simulink model "RadSimulink"  (R2020a)
settings: Solver=VariableStepAuto  StartTime=0.0  StopTime=10.0  RelTol=1e-3
values from neighbouring files (symbols this model uses):
  cz = str2num(get(handles.edit2,'string'))    [GUI.m]
  pz = str2num(get(handles.edit1,'string'))    [GUI.m]
  ti = str2num(get(handles.edit5,'string'))    [GUI.m]
  tp = str2num(get(handles.edit4,'string'))    [GUI.m]
  zl = str2num(get(handles.edit3,'string'))    [GUI.m]
libraries: neural x206, fuzblock x2
(part 2 of 3)

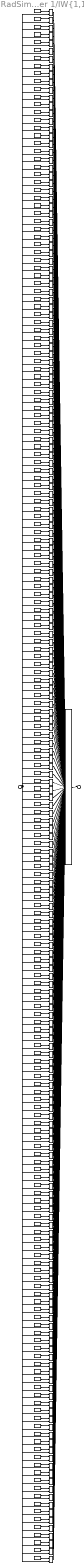
== system RadSimulink/Function Fitting Neural Network/Layer 1/IW{1,1} ==
  "pd{1,1}" : Inport  PortDimensions=5
      mask Display: e = 0.06;c1 = [120 230 180]/255;c2 = ([120 230 180]+0)/(256+128);c3 = ([120 230 180]+128)/(256+128);patch([0 1 1 0],[0 0 1 1],c1);patch([0 1 1 1-e 1-e 0+e],[0 0 1 1-e 0+e 0+e],c2);patch([0 0 1 1-e 0+e 0+e],[0 1 1 1-e 1-e 0+e],c3);plot([0 1 1 0 0],[0 0 1 1 0]);
  "IW{1,1}(1,:)'" : Constant  Value=[-1.1024971237361669285093057624180801212787628173828125;-2.42025893729763996731207953416742384433746337890625;-0.1951758632417351646548553389948210678994655609130859375;-1.7662876637968849546922456283937208354473114013671875;-2.01734664909667760213096698862500488758087158203125]
      mask Display: e = 0.06;c1 = [120 150 230]/255;c2 = ([120 150 230]+0)/383;c3 = ([120 150 230]+128)/383;patch([0 1 1 0],[0 0 1 1],c1);patch([0 1 1 1-e 1-e 0+e],[0 0 1 1-e 0+e 0+e],c2);patch([0 0 1 1-e 0+e 0+e],[0 1 1 1-e 1-e 0+e],c3);plot([0 1 1 0 0],[0 0 1 1 0]);disp('Weights');
  "IW{1,1}(10,:)'" : Constant  Value=[2.101523545932024727989073653589002788066864013671875;-1.7279665023119312738941744100884534418582916259765625;1.1178691452224647218116615476901642978191375732421875;-0.27934657220397907106956836287281475961208343505859375;2.880254256165533544020718181855045258998870849609375]
      mask Display: e = 0.06;c1 = [120 150 230]/255;c2 = ([120 150 230]+0)/383;c3 = ([120 150 230]+128)/383;patch([0 1 1 0],[0 0 1 1],c1);patch([0 1 1 1-e 1-e 0+e],[0 0 1 1-e 0+e 0+e],c2);patch([0 0 1 1-e 0+e 0+e],[0 1 1 1-e 1-e 0+e],c3);plot([0 1 1 0 0],[0 0 1 1 0]);disp('Weights');
  "IW{1,1}(100,:)'" : Constant  Value=[-1.0080768381000433375760394483222626149654388427734375;0.06504466674938051695686880293578724376857280731201171875;-2.437083695314801179421237975475378334522247314453125;-0.60085262232023317618967439557309262454509735107421875;2.912213889031785907235416743787936866283416748046875]
      mask Display: e = 0.06;c1 = [120 150 230]/255;c2 = ([120 150 230]+0)/383;c3 = ([120 150 230]+128)/383;patch([0 1 1 0],[0 0 1 1],c1);patch([0 1 1 1-e 1-e 0+e],[0 0 1 1-e 0+e 0+e],c2);patch([0 0 1 1-e 0+e 0+e],[0 1 1 1-e 1-e 0+e],c3);plot([0 1 1 0 0],[0 0 1 1 0]);disp('Weights');
  "IW{1,1}(101,:)'" : Constant  Value=[1.90336093057931687866357606253586709499359130859375;-1.126709319667938746789559445460326969623565673828125;-2.31817597529505636799740386777557432651519775390625;1.6272516351571402193343374165124259889125823974609375;-1.368723252103397403089957151678390800952911376953125]
      mask Display: e = 0.06;c1 = [120 150 230]/255;c2 = ([120 150 230]+0)/383;c3 = ([120 150 230]+128)/383;patch([0 1 1 0],[0 0 1 1],c1);patch([0 1 1 1-e 1-e 0+e],[0 0 1 1-e 0+e 0+e],c2);patch([0 0 1 1-e 0+e 0+e],[0 1 1 1-e 1-e 0+e],c3);plot([0 1 1 0 0],[0 0 1 1 0]);disp('Weights');
  "IW{1,1}(102,:)'" : Constant  Value=[-3.420026756921864308225167405907995998859405517578125;-2.3719950536146399144854512996971607208251953125;1.1313743416636159455634924597688950598239898681640625;-0.8552105117849888582526318714371882379055023193359375;0.233304600818531604478067720265244133770465850830078125]
      mask Display: e = 0.06;c1 = [120 150 230]/255;c2 = ([120 150 230]+0)/383;c3 = ([120 150 230]+128)/383;patch([0 1 1 0],[0 0 1 1],c1);patch([0 1 1 1-e 1-e 0+e],[0 0 1 1-e 0+e 0+e],c2);patch([0 0 1 1-e 0+e 0+e],[0 1 1 1-e 1-e 0+e],c3);plot([0 1 1 0 0],[0 0 1 1 0]);disp('Weights');
  "IW{1,1}(103,:)'" : Constant  Value=[-0.7245749152369149737040743275429122149944305419921875;2.719538996825153542857833599555306136608123779296875;-0.34034567501443147019557500243536196649074554443359375;-2.62175331828034519077164077316410839557647705078125;-1.79375045778324260226099795545451343059539794921875]
      mask Display: e = 0.06;c1 = [120 150 230]/255;c2 = ([120 150 230]+0)/383;c3 = ([120 150 230]+128)/383;patch([0 1 1 0],[0 0 1 1],c1);patch([0 1 1 1-e 1-e 0+e],[0 0 1 1-e 0+e 0+e],c2);patch([0 0 1 1-e 0+e 0+e],[0 1 1 1-e 1-e 0+e],c3);plot([0 1 1 0 0],[0 0 1 1 0]);disp('Weights');
  "IW{1,1}(104,:)'" : Constant  Value=[-1.8276546952938861334558851012843661010265350341796875;3.1424452420276391961806439212523400783538818359375;2.819758895819064914434193269698880612850189208984375;-0.10000487520686705822381412644972442649304866790771484375;0.88030108858768307822373344606603495776653289794921875]
      mask Display: e = 0.06;c1 = [120 150 230]/255;c2 = ([120 150 230]+0)/383;c3 = ([120 150 230]+128)/383;patch([0 1 1 0],[0 0 1 1],c1);patch([0 1 1 1-e 1-e 0+e],[0 0 1 1-e 0+e 0+e],c2);patch([0 0 1 1-e 0+e 0+e],[0 1 1 1-e 1-e 0+e],c3);plot([0 1 1 0 0],[0 0 1 1 0]);disp('Weights');
  "IW{1,1}(105,:)'" : Constant  Value=[-1.955119046550140016194063719012774527072906494140625;2.26029192919587718080265403841622173786163330078125;-0.84774494451610082901282794409780763089656829833984375;-0.38953484467059806828359569408348761498928070068359375;2.197168941225040583731242804788053035736083984375]
      mask Display: e = 0.06;c1 = [120 150 230]/255;c2 = ([120 150 230]+0)/383;c3 = ([120 150 230]+128)/383;patch([0 1 1 0],[0 0 1 1],c1);patch([0 1 1 1-e 1-e 0+e],[0 0 1 1-e 0+e 0+e],c2);patch([0 0 1 1-e 0+e 0+e],[0 1 1 1-e 1-e 0+e],c3);plot([0 1 1 0 0],[0 0 1 1 0]);disp('Weights');
  "IW{1,1}(106,:)'" : Constant  Value=[-2.32279050408599641031059945817105472087860107421875;0.94744858728796532698623877877253107726573944091796875;-1.5499805306115224112772921216674149036407470703125;2.097487556649907158856649402878247201442718505859375;-1.791807377519587074488072175881825387477874755859375]
      mask Display: e = 0.06;c1 = [120 150 230]/255;c2 = ([120 150 230]+0)/383;c3 = ([120 150 230]+128)/383;patch([0 1 1 0],[0 0 1 1],c1);patch([0 1 1 1-e 1-e 0+e],[0 0 1 1-e 0+e 0+e],c2);patch([0 0 1 1-e 0+e 0+e],[0 1 1 1-e 1-e 0+e],c3);plot([0 1 1 0 0],[0 0 1 1 0]);disp('Weights');
  "IW{1,1}(107,:)'" : Constant  Value=[1.1809257823517860241935295562143437564373016357421875;-2.377719411022709561365218178252689540386199951171875;0.2141296858350458520714454380140523426234722137451171875;-1.1815675916247567744932212008279748260974884033203125;2.70168779430114813777663584914989769458770751953125]
      mask Display: e = 0.06;c1 = [120 150 230]/255;c2 = ([120 150 230]+0)/383;c3 = ([120 150 230]+128)/383;patch([0 1 1 0],[0 0 1 1],c1);patch([0 1 1 1-e 1-e 0+e],[0 0 1 1-e 0+e 0+e],c2);patch([0 0 1 1-e 0+e 0+e],[0 1 1 1-e 1-e 0+e],c3);plot([0 1 1 0 0],[0 0 1 1 0]);disp('Weights');
  "IW{1,1}(108,:)'" : Constant  Value=[-1.754914904257402152865097377798520028591156005859375;-2.0911361399005361505487599060870707035064697265625;2.542284700714983358693643822334706783294677734375;1.9958867986801454019740731382626108825206756591796875;-1.67034476062302683629923194530420005321502685546875]
      mask Display: e = 0.06;c1 = [120 150 230]/255;c2 = ([120 150 230]+0)/383;c3 = ([120 150 230]+128)/383;patch([0 1 1 0],[0 0 1 1],c1);patch([0 1 1 1-e 1-e 0+e],[0 0 1 1-e 0+e 0+e],c2);patch([0 0 1 1-e 0+e 0+e],[0 1 1 1-e 1-e 0+e],c3);plot([0 1 1 0 0],[0 0 1 1 0]);disp('Weights');
  "IW{1,1}(109,:)'" : Constant  Value=[0.956521745717475280201824716641567647457122802734375;-2.50335089270634636449130994151346385478973388671875;1.2037065443916625806508591267629526555538177490234375;0.60555610759611766535925880816648714244365692138671875;-2.731580459628556667439625016413629055023193359375]
      mask Display: e = 0.06;c1 = [120 150 230]/255;c2 = ([120 150 230]+0)/383;c3 = ([120 150 230]+128)/383;patch([0 1 1 0],[0 0 1 1],c1);patch([0 1 1 1-e 1-e 0+e],[0 0 1 1-e 0+e 0+e],c2);patch([0 0 1 1-e 0+e 0+e],[0 1 1 1-e 1-e 0+e],c3);plot([0 1 1 0 0],[0 0 1 1 0]);disp('Weights');
  "IW{1,1}(11,:)'" : Constant  Value=[-2.907949635275226540898074745200574398040771484375;1.1530656903068148277924365174840204417705535888671875;-0.443569230139339631957540177609189413487911224365234375;1.4059497597816703606810051496722735464572906494140625;2.099149397548405460156573099084198474884033203125]
      mask Display: e = 0.06;c1 = [120 150 230]/255;c2 = ([120 150 230]+0)/383;c3 = ([120 150 230]+128)/383;patch([0 1 1 0],[0 0 1 1],c1);patch([0 1 1 1-e 1-e 0+e],[0 0 1 1-e 0+e 0+e],c2);patch([0 0 1 1-e 0+e 0+e],[0 1 1 1-e 1-e 0+e],c3);plot([0 1 1 0 0],[0 0 1 1 0]);disp('Weights');
  "IW{1,1}(110,:)'" : Constant  Value=[-1.6020415711927344926124305857229046523571014404296875;-3.0917400563691845860603280016221106052398681640625;-0.9714288758683198299337391290464438498020172119140625;-2.2679764643333104601197192096151411533355712890625;0.669326600522941905779816806898452341556549072265625]
      mask Display: e = 0.06;c1 = [120 150 230]/255;c2 = ([120 150 230]+0)/383;c3 = ([120 150 230]+128)/383;patch([0 1 1 0],[0 0 1 1],c1);patch([0 1 1 1-e 1-e 0+e],[0 0 1 1-e 0+e 0+e],c2);patch([0 0 1 1-e 0+e 0+e],[0 1 1 1-e 1-e 0+e],c3);plot([0 1 1 0 0],[0 0 1 1 0]);disp('Weights');
  "IW{1,1}(111,:)'" : Constant  Value=[1.162354455160433897020766380592249333858489990234375;1.5263583187996536683073145468370057642459869384765625;-1.9318884103074271951783202894148416817188262939453125;-1.7446165484139708468092067050747573375701904296875;-2.8400204539045343921088715433143079280853271484375]
      mask Display: e = 0.06;c1 = [120 150 230]/255;c2 = ([120 150 230]+0)/383;c3 = ([120 150 230]+128)/383;patch([0 1 1 0],[0 0 1 1],c1);patch([0 1 1 1-e 1-e 0+e],[0 0 1 1-e 0+e 0+e],c2);patch([0 0 1 1-e 0+e 0+e],[0 1 1 1-e 1-e 0+e],c3);plot([0 1 1 0 0],[0 0 1 1 0]);disp('Weights');
  "IW{1,1}(112,:)'" : Constant  Value=[0.66765089953219725060762357315979897975921630859375;-1.9914835830233432734104326300439424812793731689453125;1.8164696639128068422763817579834721982479095458984375;0.2068577426128505869495910474142874591052532196044921875;-3.01193773462074698699098007637076079845428466796875]
      mask Display: e = 0.06;c1 = [120 150 230]/255;c2 = ([120 150 230]+0)/383;c3 = ([120 150 230]+128)/383;patch([0 1 1 0],[0 0 1 1],c1);patch([0 1 1 1-e 1-e 0+e],[0 0 1 1-e 0+e 0+e],c2);patch([0 0 1 1-e 0+e 0+e],[0 1 1 1-e 1-e 0+e],c3);plot([0 1 1 0 0],[0 0 1 1 0]);disp('Weights');
  "IW{1,1}(113,:)'" : Constant  Value=[-1.3410265394460332277759562202845700085163116455078125;1.4528723409373867081484377195010893046855926513671875;4.09747304901806597143831822904758155345916748046875;0.5194580229380536540162438541301526129245758056640625;1.6134633116029968302740371655090712010860443115234375]
      mask Display: e = 0.06;c1 = [120 150 230]/255;c2 = ([120 150 230]+0)/383;c3 = ([120 150 230]+128)/383;patch([0 1 1 0],[0 0 1 1],c1);patch([0 1 1 1-e 1-e 0+e],[0 0 1 1-e 0+e 0+e],c2);patch([0 0 1 1-e 0+e 0+e],[0 1 1 1-e 1-e 0+e],c3);plot([0 1 1 0 0],[0 0 1 1 0]);disp('Weights');
  "IW{1,1}(114,:)'" : Constant  Value=[2.19775277811335367772471727221272885799407958984375;1.530445614021247013880611120839603245258331298828125;-0.51276813648967511927168061447446234524250030517578125;-1.439648029384903882288426757440902292728424072265625;-3.040338611642841026849737318116240203380584716796875]
      mask Display: e = 0.06;c1 = [120 150 230]/255;c2 = ([120 150 230]+0)/383;c3 = ([120 150 230]+128)/383;patch([0 1 1 0],[0 0 1 1],c1);patch([0 1 1 1-e 1-e 0+e],[0 0 1 1-e 0+e 0+e],c2);patch([0 0 1 1-e 0+e 0+e],[0 1 1 1-e 1-e 0+e],c3);plot([0 1 1 0 0],[0 0 1 1 0]);disp('Weights');
  "IW{1,1}(115,:)'" : Constant  Value=[1.8961919249288563538158314258907921612262725830078125;0.41129351010530157406464013547520153224468231201171875;-2.248095539210364979254563877475447952747344970703125;-1.3547463652555962188017701919307000935077667236328125;2.75720385899369802018554764799773693084716796875]
      mask Display: e = 0.06;c1 = [120 150 230]/255;c2 = ([120 150 230]+0)/383;c3 = ([120 150 230]+128)/383;patch([0 1 1 0],[0 0 1 1],c1);patch([0 1 1 1-e 1-e 0+e],[0 0 1 1-e 0+e 0+e],c2);patch([0 0 1 1-e 0+e 0+e],[0 1 1 1-e 1-e 0+e],c3);plot([0 1 1 0 0],[0 0 1 1 0]);disp('Weights');
  "IW{1,1}(116,:)'" : Constant  Value=[2.954413030926638317197330252383835613727569580078125;-0.88633584372641716075946760611259378492832183837890625;-2.12033955906994986406743919360451400279998779296875;1.76130835936309804168331538676284253597259521484375;-0.1357983118735323901926648204607772640883922576904296875]
      mask Display: e = 0.06;c1 = [120 150 230]/255;c2 = ([120 150 230]+0)/383;c3 = ([120 150 230]+128)/383;patch([0 1 1 0],[0 0 1 1],c1);patch([0 1 1 1-e 1-e 0+e],[0 0 1 1-e 0+e 0+e],c2);patch([0 0 1 1-e 0+e 0+e],[0 1 1 1-e 1-e 0+e],c3);plot([0 1 1 0 0],[0 0 1 1 0]);disp('Weights');
  "IW{1,1}(117,:)'" : Constant  Value=[-4.02991069960216474754588489304296672344207763671875;1.9833370043181337560866950298077426850795745849609375;0.046775997960406622000473220168714760802686214447021484375;0.734776445964431701440844335593283176422119140625;-0.89640460868724025633724750150577165186405181884765625]
      mask Display: e = 0.06;c1 = [120 150 230]/255;c2 = ([120 150 230]+0)/383;c3 = ([120 150 230]+128)/383;patch([0 1 1 0],[0 0 1 1],c1);patch([0 1 1 1-e 1-e 0+e],[0 0 1 1-e 0+e 0+e],c2);patch([0 0 1 1-e 0+e 0+e],[0 1 1 1-e 1-e 0+e],c3);plot([0 1 1 0 0],[0 0 1 1 0]);disp('Weights');
  "IW{1,1}(118,:)'" : Constant  Value=[0.69244616119575308488265363848768174648284912109375;-1.6956716845926533832056293249479494988918304443359375;-2.57710351212775901075247020344249904155731201171875;-2.702734985715044668808104688650928437709808349609375;1.1181759860109174997688796793227083981037139892578125]
      mask Display: e = 0.06;c1 = [120 150 230]/255;c2 = ([120 150 230]+0)/383;c3 = ([120 150 230]+128)/383;patch([0 1 1 0],[0 0 1 1],c1);patch([0 1 1 1-e 1-e 0+e],[0 0 1 1-e 0+e 0+e],c2);patch([0 0 1 1-e 0+e 0+e],[0 1 1 1-e 1-e 0+e],c3);plot([0 1 1 0 0],[0 0 1 1 0]);disp('Weights');
  "IW{1,1}(119,:)'" : Constant  Value=[-2.737537295445146678929404515656642615795135498046875;-0.81241155860551350631482137032435275614261627197265625;-1.0933153794961827376397422995069064199924468994140625;1.143052193414451966901879131910391151905059814453125;2.879019332145628329300279801827855408191680908203125]
      mask Display: e = 0.06;c1 = [120 150 230]/255;c2 = ([120 150 230]+0)/383;c3 = ([120 150 230]+128)/383;patch([0 1 1 0],[0 0 1 1],c1);patch([0 1 1 1-e 1-e 0+e],[0 0 1 1-e 0+e 0+e],c2);patch([0 0 1 1-e 0+e 0+e],[0 1 1 1-e 1-e 0+e],c3);plot([0 1 1 0 0],[0 0 1 1 0]);disp('Weights');
  "IW{1,1}(12,:)'" : Constant  Value=[-1.8135943539993935047505146940238773822784423828125;-3.103634828364266073918997790315188467502593994140625;-0.301922130932056387297990340812248177826404571533203125;-0.1237979411920113459455450310997548513114452362060546875;-1.41910702071063798967998081934638321399688720703125]
      mask Display: e = 0.06;c1 = [120 150 230]/255;c2 = ([120 150 230]+0)/383;c3 = ([120 150 230]+128)/383;patch([0 1 1 0],[0 0 1 1],c1);patch([0 1 1 1-e 1-e 0+e],[0 0 1 1-e 0+e 0+e],c2);patch([0 0 1 1-e 0+e 0+e],[0 1 1 1-e 1-e 0+e],c3);plot([0 1 1 0 0],[0 0 1 1 0]);disp('Weights');
  "IW{1,1}(120,:)'" : Constant  Value=[-3.34213975887307146450666550663299858570098876953125;2.790486751775154150578828193829394876956939697265625;-0.302405210762672016500118843396194279193878173828125;-0.257404953550620929636494338410557247698307037353515625;-0.2017369321757929989669122505802079103887081146240234375]
      mask Display: e = 0.06;c1 = [120 150 230]/255;c2 = ([120 150 230]+0)/383;c3 = ([120 150 230]+128)/383;patch([0 1 1 0],[0 0 1 1],c1);patch([0 1 1 1-e 1-e 0+e],[0 0 1 1-e 0+e 0+e],c2);patch([0 0 1 1-e 0+e 0+e],[0 1 1 1-e 1-e 0+e],c3);plot([0 1 1 0 0],[0 0 1 1 0]);disp('Weights');
  "IW{1,1}(121,:)'" : Constant  Value=[-3.392294521732422740711854203254915773868560791015625;0.20942239687643027234997816776740364730358123779296875;-1.3125370002407936720345560388523153960704803466796875;-0.14378919640720833061919847750687040388584136962890625;2.228432434247277882377602509222924709320068359375]
      mask Display: e = 0.06;c1 = [120 150 230]/255;c2 = ([120 150 230]+0)/383;c3 = ([120 150 230]+128)/383;patch([0 1 1 0],[0 0 1 1],c1);patch([0 1 1 1-e 1-e 0+e],[0 0 1 1-e 0+e 0+e],c2);patch([0 0 1 1-e 0+e 0+e],[0 1 1 1-e 1-e 0+e],c3);plot([0 1 1 0 0],[0 0 1 1 0]);disp('Weights');
  "IW{1,1}(122,:)'" : Constant  Value=[-1.75905539540671629339385617640800774097442626953125;-3.187451027508598766502245780429802834987640380859375;-1.645529519450947386616235235123895108699798583984375;2.67049482505225466155707181314937770366668701171875;0.7503515450185374024982820628792978823184967041015625]
      mask Display: e = 0.06;c1 = [120 150 230]/255;c2 = ([120 150 230]+0)/383;c3 = ([120 150 230]+128)/383;patch([0 1 1 0],[0 0 1 1],c1);patch([0 1 1 1-e 1-e 0+e],[0 0 1 1-e 0+e 0+e],c2);patch([0 0 1 1-e 0+e 0+e],[0 1 1 1-e 1-e 0+e],c3);plot([0 1 1 0 0],[0 0 1 1 0]);disp('Weights');
  "IW{1,1}(123,:)'" : Constant  Value=[-2.788792847496659899064752607955597341060638427734375;1.6776656245569110392779066387447528541088104248046875;-0.304824112680752212778401144532836042344570159912109375;-1.2160626373394511912096049854881130158901214599609375;2.776459447970099692071244135149754583835601806640625]
      mask Display: e = 0.06;c1 = [120 150 230]/255;c2 = ([120 150 230]+0)/383;c3 = ([120 150 230]+128)/383;patch([0 1 1 0],[0 0 1 1],c1);patch([0 1 1 1-e 1-e 0+e],[0 0 1 1-e 0+e 0+e],c2);patch([0 0 1 1-e 0+e 0+e],[0 1 1 1-e 1-e 0+e],c3);plot([0 1 1 0 0],[0 0 1 1 0]);disp('Weights');
  "IW{1,1}(124,:)'" : Constant  Value=[-0.80664229937318487895225871397997252643108367919921875;-2.19903462899787793816130943014286458492279052734375;-1.4063350337747901885876444794121198356151580810546875;-2.9997677450250908037787667126394808292388916015625;0.331515823929653230539571495683048851788043975830078125]
      mask Display: e = 0.06;c1 = [120 150 230]/255;c2 = ([120 150 230]+0)/383;c3 = ([120 150 230]+128)/383;patch([0 1 1 0],[0 0 1 1],c1);patch([0 1 1 1-e 1-e 0+e],[0 0 1 1-e 0+e 0+e],c2);patch([0 0 1 1-e 0+e 0+e],[0 1 1 1-e 1-e 0+e],c3);plot([0 1 1 0 0],[0 0 1 1 0]);disp('Weights');
  "IW{1,1}(125,:)'" : Constant  Value=[-1.2121170429702983195596743826172314584255218505859375;2.16495630448694864611525190412066876888275146484375;-2.124413283432712962195410000276751816272735595703125;-2.12457525827358661985044818720780313014984130859375;-0.67667681596699591484167513044667430222034454345703125]
      mask Display: e = 0.06;c1 = [120 150 230]/255;c2 = ([120 150 230]+0)/383;c3 = ([120 150 230]+128)/383;patch([0 1 1 0],[0 0 1 1],c1);patch([0 1 1 1-e 1-e 0+e],[0 0 1 1-e 0+e 0+e],c2);patch([0 0 1 1-e 0+e 0+e],[0 1 1 1-e 1-e 0+e],c3);plot([0 1 1 0 0],[0 0 1 1 0]);disp('Weights');
  "IW{1,1}(126,:)'" : Constant  Value=[-0.7999665946026801588430998890544287860393524169921875;-2.048714130895408658261658274568617343902587890625;1.4521789817209083128801694329013116657733917236328125;0.9816305616312812620805061669670976698398590087890625;3.159907850832450293410147423855960369110107421875]
      mask Display: e = 0.06;c1 = [120 150 230]/255;c2 = ([120 150 230]+0)/383;c3 = ([120 150 230]+128)/383;patch([0 1 1 0],[0 0 1 1],c1);patch([0 1 1 1-e 1-e 0+e],[0 0 1 1-e 0+e 0+e],c2);patch([0 0 1 1-e 0+e 0+e],[0 1 1 1-e 1-e 0+e],c3);plot([0 1 1 0 0],[0 0 1 1 0]);disp('Weights');
  "IW{1,1}(127,:)'" : Constant  Value=[-0.369712940205680073990635037262109108269214630126953125;-2.54328278717233846606404767953790724277496337890625;-2.16124119727358987574916682206094264984130859375;-0.200046400540370095111342152449651621282100677490234375;-1.5920004911277414461068246964714489877223968505859375]
      mask Display: e = 0.06;c1 = [120 150 230]/255;c2 = ([120 150 230]+0)/383;c3 = ([120 150 230]+128)/383;patch([0 1 1 0],[0 0 1 1],c1);patch([0 1 1 1-e 1-e 0+e],[0 0 1 1-e 0+e 0+e],c2);patch([0 0 1 1-e 0+e 0+e],[0 1 1 1-e 1-e 0+e],c3);plot([0 1 1 0 0],[0 0 1 1 0]);disp('Weights');
  "IW{1,1}(128,:)'" : Constant  Value=[0.461335917378665083532496282714419066905975341796875;-2.6164804216071484432859506341628730297088623046875;1.652166158439022591863931666011922061443328857421875;2.589731154281836200681254922528751194477081298828125;1.3217704781755070797544249217025935649871826171875]
      mask Display: e = 0.06;c1 = [120 150 230]/255;c2 = ([120 150 230]+0)/383;c3 = ([120 150 230]+128)/383;patch([0 1 1 0],[0 0 1 1],c1);patch([0 1 1 1-e 1-e 0+e],[0 0 1 1-e 0+e 0+e],c2);patch([0 0 1 1-e 0+e 0+e],[0 1 1 1-e 1-e 0+e],c3);plot([0 1 1 0 0],[0 0 1 1 0]);disp('Weights');
  "IW{1,1}(129,:)'" : Constant  Value=[2.06883163379194723319187687593512237071990966796875;1.80290688565839207768704000045545399188995361328125;-0.72578536253818415335814506761380471289157867431640625;-2.928418897294223111060773589997552335262298583984375;2.406764656464925877799032605253159999847412109375]
      mask Display: e = 0.06;c1 = [120 150 230]/255;c2 = ([120 150 230]+0)/383;c3 = ([120 150 230]+128)/383;patch([0 1 1 0],[0 0 1 1],c1);patch([0 1 1 1-e 1-e 0+e],[0 0 1 1-e 0+e 0+e],c2);patch([0 0 1 1-e 0+e 0+e],[0 1 1 1-e 1-e 0+e],c3);plot([0 1 1 0 0],[0 0 1 1 0]);disp('Weights');
  "IW{1,1}(13,:)'" : Constant  Value=[-1.8300328795259355185720551162376068532466888427734375;-1.11629153957151938669767332612536847591400146484375;1.721749848709251740075387715478427708148956298828125;2.704650039807795725010919341002590954303741455078125;1.09610543472943700038513270555995404720306396484375]
      mask Display: e = 0.06;c1 = [120 150 230]/255;c2 = ([120 150 230]+0)/383;c3 = ([120 150 230]+128)/383;patch([0 1 1 0],[0 0 1 1],c1);patch([0 1 1 1-e 1-e 0+e],[0 0 1 1-e 0+e 0+e],c2);patch([0 0 1 1-e 0+e 0+e],[0 1 1 1-e 1-e 0+e],c3);plot([0 1 1 0 0],[0 0 1 1 0]);disp('Weights');
  "IW{1,1}(130,:)'" : Constant  Value=[-1.928829470017271230375399682088755071163177490234375;2.64991828479049384981180992326699197292327880859375;-1.2320867205501879748652527268859557807445526123046875;-1.05303592762808317928602264146320521831512451171875;-1.8733227480287795163604869230766780674457550048828125]
      mask Display: e = 0.06;c1 = [120 150 230]/255;c2 = ([120 150 230]+0)/383;c3 = ([120 150 230]+128)/383;patch([0 1 1 0],[0 0 1 1],c1);patch([0 1 1 1-e 1-e 0+e],[0 0 1 1-e 0+e 0+e],c2);patch([0 0 1 1-e 0+e 0+e],[0 1 1 1-e 1-e 0+e],c3);plot([0 1 1 0 0],[0 0 1 1 0]);disp('Weights');
  "IW{1,1}(131,:)'" : Constant  Value=[2.07505260176850558906380683765746653079986572265625;1.76758288123504758715398565982468426227569580078125;2.101289526858626022232101604458875954151153564453125;1.074093081223086443287684232927858829498291015625;2.2848854964617668628079627524130046367645263671875]
      mask Display: e = 0.06;c1 = [120 150 230]/255;c2 = ([120 150 230]+0)/383;c3 = ([120 150 230]+128)/383;patch([0 1 1 0],[0 0 1 1],c1);patch([0 1 1 1-e 1-e 0+e],[0 0 1 1-e 0+e 0+e],c2);patch([0 0 1 1-e 0+e 0+e],[0 1 1 1-e 1-e 0+e],c3);plot([0 1 1 0 0],[0 0 1 1 0]);disp('Weights');
  "IW{1,1}(132,:)'" : Constant  Value=[1.7657805278861296027770322325523011386394500732421875;1.9688266499752717919591304962523281574249267578125;1.6354915842362334199577844628947786986827850341796875;-2.4718935657278731099495416856370866298675537109375;1.20631616848982314849081376451067626476287841796875]
      mask Display: e = 0.06;c1 = [120 150 230]/255;c2 = ([120 150 230]+0)/383;c3 = ([120 150 230]+128)/383;patch([0 1 1 0],[0 0 1 1],c1);patch([0 1 1 1-e 1-e 0+e],[0 0 1 1-e 0+e 0+e],c2);patch([0 0 1 1-e 0+e 0+e],[0 1 1 1-e 1-e 0+e],c3);plot([0 1 1 0 0],[0 0 1 1 0]);disp('Weights');
  "IW{1,1}(133,:)'" : Constant  Value=[1.67679621443762361110429992550052702426910400390625;2.371141874793253112585489361663348972797393798828125;-1.7217387947356572741597346976050175726413726806640625;2.125150756548237040988169610500335693359375;-0.436648609803640674886793249243055470287799835205078125]
      mask Display: e = 0.06;c1 = [120 150 230]/255;c2 = ([120 150 230]+0)/383;c3 = ([120 150 230]+128)/383;patch([0 1 1 0],[0 0 1 1],c1);patch([0 1 1 1-e 1-e 0+e],[0 0 1 1-e 0+e 0+e],c2);patch([0 0 1 1-e 0+e 0+e],[0 1 1 1-e 1-e 0+e],c3);plot([0 1 1 0 0],[0 0 1 1 0]);disp('Weights');
  "IW{1,1}(134,:)'" : Constant  Value=[-2.73630229716275952256410164409317076206207275390625;-0.480445149051417830232679762048064731061458587646484375;-3.521201645905150723336873852531425654888153076171875;0.6171924277463134433929781152983196079730987548828125;-0.2089751766994900616936092774267308413982391357421875]
      mask Display: e = 0.06;c1 = [120 150 230]/255;c2 = ([120 150 230]+0)/383;c3 = ([120 150 230]+128)/383;patch([0 1 1 0],[0 0 1 1],c1);patch([0 1 1 1-e 1-e 0+e],[0 0 1 1-e 0+e 0+e],c2);patch([0 0 1 1-e 0+e 0+e],[0 1 1 1-e 1-e 0+e],c3);plot([0 1 1 0 0],[0 0 1 1 0]);disp('Weights');
  "IW{1,1}(135,:)'" : Constant  Value=[-2.092920957633349843263204093091189861297607421875;1.489563112900500474466980449506081640720367431640625;-1.7361528232531229232193936695693992078304290771484375;1.8345350758822103198752984098973684012889862060546875;2.04631108625287794211544678546488285064697265625]
      mask Display: e = 0.06;c1 = [120 150 230]/255;c2 = ([120 150 230]+0)/383;c3 = ([120 150 230]+128)/383;patch([0 1 1 0],[0 0 1 1],c1);patch([0 1 1 1-e 1-e 0+e],[0 0 1 1-e 0+e 0+e],c2);patch([0 0 1 1-e 0+e 0+e],[0 1 1 1-e 1-e 0+e],c3);plot([0 1 1 0 0],[0 0 1 1 0]);disp('Weights');
  "IW{1,1}(136,:)'" : Constant  Value=[0.99821225273482327988716633626609109342098236083984375;-0.6539734250895532507996676940820179879665374755859375;1.6239471314550166791690344325616024434566497802734375;1.26520374508919530853745527565479278564453125;3.719149472968293679286944097839295864105224609375]
      mask Display: e = 0.06;c1 = [120 150 230]/255;c2 = ([120 150 230]+0)/383;c3 = ([120 150 230]+128)/383;patch([0 1 1 0],[0 0 1 1],c1);patch([0 1 1 1-e 1-e 0+e],[0 0 1 1-e 0+e 0+e],c2);patch([0 0 1 1-e 0+e 0+e],[0 1 1 1-e 1-e 0+e],c3);plot([0 1 1 0 0],[0 0 1 1 0]);disp('Weights');
  "IW{1,1}(137,:)'" : Constant  Value=[1.09921092338686587908114233869127929210662841796875;1.9587283678469706860170163054135628044605255126953125;1.7064523739663155499357571898144669830799102783203125;-2.25686929444278394640832630102522671222686767578125;1.1589095167163296906664982088841497898101806640625]
      mask Display: e = 0.06;c1 = [120 150 230]/255;c2 = ([120 150 230]+0)/383;c3 = ([120 150 230]+128)/383;patch([0 1 1 0],[0 0 1 1],c1);patch([0 1 1 1-e 1-e 0+e],[0 0 1 1-e 0+e 0+e],c2);patch([0 0 1 1-e 0+e 0+e],[0 1 1 1-e 1-e 0+e],c3);plot([0 1 1 0 0],[0 0 1 1 0]);disp('Weights');
  "IW{1,1}(138,:)'" : Constant  Value=[-2.173089817476193896794711690745316445827484130859375;-2.954055404105415671978107639006339013576507568359375;0.079718393381679353293378653688705526292324066162109375;-1.0080231626911455578010645695030689239501953125;-0.64648656741367716005441934612463228404521942138671875]
      mask Display: e = 0.06;c1 = [120 150 230]/255;c2 = ([120 150 230]+0)/383;c3 = ([120 150 230]+128)/383;patch([0 1 1 0],[0 0 1 1],c1);patch([0 1 1 1-e 1-e 0+e],[0 0 1 1-e 0+e 0+e],c2);patch([0 0 1 1-e 0+e 0+e],[0 1 1 1-e 1-e 0+e],c3);plot([0 1 1 0 0],[0 0 1 1 0]);disp('Weights');
  "IW{1,1}(139,:)'" : Constant  Value=[-1.5916282796347764882938236041809432208538055419921875;2.0757580463283371585703207529149949550628662109375;-1.510034253207589660661369634908623993396759033203125;-1.4244032926568517272158942432724870741367340087890625;-1.8896287868978240975792459721560589969158172607421875]
      mask Display: e = 0.06;c1 = [120 150 230]/255;c2 = ([120 150 230]+0)/383;c3 = ([120 150 230]+128)/383;patch([0 1 1 0],[0 0 1 1],c1);patch([0 1 1 1-e 1-e 0+e],[0 0 1 1-e 0+e 0+e],c2);patch([0 0 1 1-e 0+e 0+e],[0 1 1 1-e 1-e 0+e],c3);plot([0 1 1 0 0],[0 0 1 1 0]);disp('Weights');
  "IW{1,1}(14,:)'" : Constant  Value=[-2.758905414668205491324215472559444606304168701171875;0.768267786076949565909899320104159414768218994140625;1.7894579207928626995993681703112088143825531005859375;-0.88373056094076141153692560692434199154376983642578125;-2.146474138287855826234817868680693209171295166015625]
      mask Display: e = 0.06;c1 = [120 150 230]/255;c2 = ([120 150 230]+0)/383;c3 = ([120 150 230]+128)/383;patch([0 1 1 0],[0 0 1 1],c1);patch([0 1 1 1-e 1-e 0+e],[0 0 1 1-e 0+e 0+e],c2);patch([0 0 1 1-e 0+e 0+e],[0 1 1 1-e 1-e 0+e],c3);plot([0 1 1 0 0],[0 0 1 1 0]);disp('Weights');
  "IW{1,1}(140,:)'" : Constant  Value=[2.271076125176052951104566091089509427547454833984375;2.09703819092209098329249172820709645748138427734375;4.0616776154045783897572619025595486164093017578125;2.49263816796556003652085564681328833103179931640625;2.23933569557349176903926490922458469867706298828125]
      mask Display: e = 0.06;c1 = [120 150 230]/255;c2 = ([120 150 230]+0)/383;c3 = ([120 150 230]+128)/383;patch([0 1 1 0],[0 0 1 1],c1);patch([0 1 1 1-e 1-e 0+e],[0 0 1 1-e 0+e 0+e],c2);patch([0 0 1 1-e 0+e 0+e],[0 1 1 1-e 1-e 0+e],c3);plot([0 1 1 0 0],[0 0 1 1 0]);disp('Weights');
  "IW{1,1}(141,:)'" : Constant  Value=[1.6504413640252832973231988944462500512599945068359375;-1.047315279243952179655252621159888803958892822265625;2.241708705851370719841497702873311936855316162109375;-2.590955267060750966123805483221076428890228271484375;0.21851270777601639050402582142851315438747406005859375]
      mask Display: e = 0.06;c1 = [120 150 230]/255;c2 = ([120 150 230]+0)/383;c3 = ([120 150 230]+128)/383;patch([0 1 1 0],[0 0 1 1],c1);patch([0 1 1 1-e 1-e 0+e],[0 0 1 1-e 0+e 0+e],c2);patch([0 0 1 1-e 0+e 0+e],[0 1 1 1-e 1-e 0+e],c3);plot([0 1 1 0 0],[0 0 1 1 0]);disp('Weights');
  "IW{1,1}(142,:)'" : Constant  Value=[2.817884027792603607309729341068305075168609619140625;0.436035082331104828501366910131764598190784454345703125;-2.32635827507685188919595020706765353679656982421875;1.4162784146617897196307467311271466314792633056640625;-1.2104698007519434366230370869743637740612030029296875]
      mask Display: e = 0.06;c1 = [120 150 230]/255;c2 = ([120 150 230]+0)/383;c3 = ([120 150 230]+128)/383;patch([0 1 1 0],[0 0 1 1],c1);patch([0 1 1 1-e 1-e 0+e],[0 0 1 1-e 0+e 0+e],c2);patch([0 0 1 1-e 0+e 0+e],[0 1 1 1-e 1-e 0+e],c3);plot([0 1 1 0 0],[0 0 1 1 0]);disp('Weights');
  "IW{1,1}(143,:)'" : Constant  Value=[-2.390922879471835127418444244540296494960784912109375;-1.15395377483196970302969930344261229038238525390625;2.148487360703988269250430676038376986980438232421875;-0.10042043934661648574291348268161527812480926513671875;2.179134051723498277652879551169462502002716064453125]
      mask Display: e = 0.06;c1 = [120 150 230]/255;c2 = ([120 150 230]+0)/383;c3 = ([120 150 230]+128)/383;patch([0 1 1 0],[0 0 1 1],c1);patch([0 1 1 1-e 1-e 0+e],[0 0 1 1-e 0+e 0+e],c2);patch([0 0 1 1-e 0+e 0+e],[0 1 1 1-e 1-e 0+e],c3);plot([0 1 1 0 0],[0 0 1 1 0]);disp('Weights');
  "IW{1,1}(144,:)'" : Constant  Value=[1.78872445746774122454780808766372501850128173828125;-2.194822993970550140119257775950245559215545654296875;-1.9764651331634255360114593713660724461078643798828125;-1.4261358216418731359453886398114264011383056640625;0.98600731283835785223601533289183862507343292236328125]
      mask Display: e = 0.06;c1 = [120 150 230]/255;c2 = ([120 150 230]+0)/383;c3 = ([120 150 230]+128)/383;patch([0 1 1 0],[0 0 1 1],c1);patch([0 1 1 1-e 1-e 0+e],[0 0 1 1-e 0+e 0+e],c2);patch([0 0 1 1-e 0+e 0+e],[0 1 1 1-e 1-e 0+e],c3);plot([0 1 1 0 0],[0 0 1 1 0]);disp('Weights');
  "IW{1,1}(145,:)'" : Constant  Value=[2.720393278337019271617691629217006266117095947265625;1.217502916812140956182020090636797249317169189453125;2.784317869932919631281720285187475383281707763671875;0.4042317146449396769725126432604156434535980224609375;1.1084182342563873024943177370005287230014801025390625]
      mask Display: e = 0.06;c1 = [120 150 230]/255;c2 = ([120 150 230]+0)/383;c3 = ([120 150 230]+128)/383;patch([0 1 1 0],[0 0 1 1],c1);patch([0 1 1 1-e 1-e 0+e],[0 0 1 1-e 0+e 0+e],c2);patch([0 0 1 1-e 0+e 0+e],[0 1 1 1-e 1-e 0+e],c3);plot([0 1 1 0 0],[0 0 1 1 0]);disp('Weights');
  "IW{1,1}(146,:)'" : Constant  Value=[-0.468636537965013866280372667461051605641841888427734375;1.3505834043433981861426218529231846332550048828125;3.016474410101753544921621141838841140270233154296875;1.7164465517066016531089189811609685420989990234375;-1.668197378707098277317300016875378787517547607421875]
      mask Display: e = 0.06;c1 = [120 150 230]/255;c2 = ([120 150 230]+0)/383;c3 = ([120 150 230]+128)/383;patch([0 1 1 0],[0 0 1 1],c1);patch([0 1 1 1-e 1-e 0+e],[0 0 1 1-e 0+e 0+e],c2);patch([0 0 1 1-e 0+e 0+e],[0 1 1 1-e 1-e 0+e],c3);plot([0 1 1 0 0],[0 0 1 1 0]);disp('Weights');
  "IW{1,1}(147,:)'" : Constant  Value=[-2.85339072465212151286095831892453134059906005859375;1.2634896291617410124530351822613738477230072021484375;0.61054150058020162372685035734320990741252899169921875;2.433585566652253451280785156995989382266998291015625;-2.211090051605514528176854582852683961391448974609375]
      mask Display: e = 0.06;c1 = [120 150 230]/255;c2 = ([120 150 230]+0)/383;c3 = ([120 150 230]+128)/383;patch([0 1 1 0],[0 0 1 1],c1);patch([0 1 1 1-e 1-e 0+e],[0 0 1 1-e 0+e 0+e],c2);patch([0 0 1 1-e 0+e 0+e],[0 1 1 1-e 1-e 0+e],c3);plot([0 1 1 0 0],[0 0 1 1 0]);disp('Weights');
  "IW{1,1}(148,:)'" : Constant  Value=[-2.722411593614745495273155029281042516231536865234375;-1.5078402626061440106042255138163454830646514892578125;-0.0628772598563666906823499402889865450561046600341796875;-1.4655233044619551119325251420377753674983978271484375;-1.9348047367618612657480525740538723766803741455078125]
      mask Display: e = 0.06;c1 = [120 150 230]/255;c2 = ([120 150 230]+0)/383;c3 = ([120 150 230]+128)/383;patch([0 1 1 0],[0 0 1 1],c1);patch([0 1 1 1-e 1-e 0+e],[0 0 1 1-e 0+e 0+e],c2);patch([0 0 1 1-e 0+e 0+e],[0 1 1 1-e 1-e 0+e],c3);plot([0 1 1 0 0],[0 0 1 1 0]);disp('Weights');
  "IW{1,1}(149,:)'" : Constant  Value=[1.5241819269484462306962768707307986915111541748046875;-1.7691581332571992835056562398676760494709014892578125;2.6235545037704266491118687554262578487396240234375;-1.263164441043074237569499018718488514423370361328125;-1.76075934947131340635451124398969113826751708984375]
      mask Display: e = 0.06;c1 = [120 150 230]/255;c2 = ([120 150 230]+0)/383;c3 = ([120 150 230]+128)/383;patch([0 1 1 0],[0 0 1 1],c1);patch([0 1 1 1-e 1-e 0+e],[0 0 1 1-e 0+e 0+e],c2);patch([0 0 1 1-e 0+e 0+e],[0 1 1 1-e 1-e 0+e],c3);plot([0 1 1 0 0],[0 0 1 1 0]);disp('Weights');
  "IW{1,1}(15,:)'" : Constant  Value=[-3.33178868023735663683737584506161510944366455078125;0.615684735613498457240666539291851222515106201171875;1.6991479271472698098222053886274807155132293701171875;-1.0998281676933554518171831659856252372264862060546875;0.873262892144545777028952215914614498615264892578125]
      mask Display: e = 0.06;c1 = [120 150 230]/255;c2 = ([120 150 230]+0)/383;c3 = ([120 150 230]+128)/383;patch([0 1 1 0],[0 0 1 1],c1);patch([0 1 1 1-e 1-e 0+e],[0 0 1 1-e 0+e 0+e],c2);patch([0 0 1 1-e 0+e 0+e],[0 1 1 1-e 1-e 0+e],c3);plot([0 1 1 0 0],[0 0 1 1 0]);disp('Weights');
  "IW{1,1}(150,:)'" : Constant  Value=[-3.385327170914499195220059846178628504276275634765625;-0.91977933088741414824340836275951005518436431884765625;-2.37360893600637634648364837630651891231536865234375;-1.01497838148896146748256796854548156261444091796875;-1.3667210636925799516205870531848631799221038818359375]
      mask Display: e = 0.06;c1 = [120 150 230]/255;c2 = ([120 150 230]+0)/383;c3 = ([120 150 230]+128)/383;patch([0 1 1 0],[0 0 1 1],c1);patch([0 1 1 1-e 1-e 0+e],[0 0 1 1-e 0+e 0+e],c2);patch([0 0 1 1-e 0+e 0+e],[0 1 1 1-e 1-e 0+e],c3);plot([0 1 1 0 0],[0 0 1 1 0]);disp('Weights');
  "IW{1,1}(151,:)'" : Constant  Value=[-0.717294192696104726536532325553707778453826904296875;-1.6434901532559018644263915120973251760005950927734375;-0.004893953778283092852230407032720904680900275707244873046875;1.6138981620547216966343739841249771416187286376953125;3.31227382259956915078191741486079990863800048828125]
      mask Display: e = 0.06;c1 = [120 150 230]/255;c2 = ([120 150 230]+0)/383;c3 = ([120 150 230]+128)/383;patch([0 1 1 0],[0 0 1 1],c1);patch([0 1 1 1-e 1-e 0+e],[0 0 1 1-e 0+e 0+e],c2);patch([0 0 1 1-e 0+e 0+e],[0 1 1 1-e 1-e 0+e],c3);plot([0 1 1 0 0],[0 0 1 1 0]);disp('Weights');
  "IW{1,1}(152,:)'" : Constant  Value=[0.56733563729477165527015358748030848801136016845703125;2.785180673334018752740348645602352917194366455078125;1.15977783202989659372406094917096197605133056640625;1.8938167299087307338112395882490091025829315185546875;-2.29403332150097671870980775565840303897857666015625]
      mask Display: e = 0.06;c1 = [120 150 230]/255;c2 = ([120 150 230]+0)/383;c3 = ([120 150 230]+128)/383;patch([0 1 1 0],[0 0 1 1],c1);patch([0 1 1 1-e 1-e 0+e],[0 0 1 1-e 0+e 0+e],c2);patch([0 0 1 1-e 0+e 0+e],[0 1 1 1-e 1-e 0+e],c3);plot([0 1 1 0 0],[0 0 1 1 0]);disp('Weights');
  "IW{1,1}(153,:)'" : Constant  Value=[2.454100154314847070935456940787844359874725341796875;1.32287701754901743100845123990438878536224365234375;0.98812621996412508540430508219287730753421783447265625;1.692680569277893898316733611864037811756134033203125;-2.1447020657619777495028756675310432910919189453125]
      mask Display: e = 0.06;c1 = [120 150 230]/255;c2 = ([120 150 230]+0)/383;c3 = ([120 150 230]+128)/383;patch([0 1 1 0],[0 0 1 1],c1);patch([0 1 1 1-e 1-e 0+e],[0 0 1 1-e 0+e 0+e],c2);patch([0 0 1 1-e 0+e 0+e],[0 1 1 1-e 1-e 0+e],c3);plot([0 1 1 0 0],[0 0 1 1 0]);disp('Weights');
  "IW{1,1}(154,:)'" : Constant  Value=[-1.8674139287858289026900138196651823818683624267578125;-1.7972669702835395444395771846757270395755767822265625;-1.8109958992713293124410256496048532426357269287109375;2.71396360376814715920090748113580048084259033203125;0.088623462346431092218068670263164676725864410400390625]
      mask Display: e = 0.06;c1 = [120 150 230]/255;c2 = ([120 150 230]+0)/383;c3 = ([120 150 230]+128)/383;patch([0 1 1 0],[0 0 1 1],c1);patch([0 1 1 1-e 1-e 0+e],[0 0 1 1-e 0+e 0+e],c2);patch([0 0 1 1-e 0+e 0+e],[0 1 1 1-e 1-e 0+e],c3);plot([0 1 1 0 0],[0 0 1 1 0]);disp('Weights');
  "IW{1,1}(155,:)'" : Constant  Value=[-1.8623544401170153417268693374353460967540740966796875;0.7449495238086385473508244103868491947650909423828125;-2.535399947195854597481456949026323854923248291015625;2.142817998177556138017507691984064877033233642578125;0.772297150263478560106022996478714048862457275390625]
      mask Display: e = 0.06;c1 = [120 150 230]/255;c2 = ([120 150 230]+0)/383;c3 = ([120 150 230]+128)/383;patch([0 1 1 0],[0 0 1 1],c1);patch([0 1 1 1-e 1-e 0+e],[0 0 1 1-e 0+e 0+e],c2);patch([0 0 1 1-e 0+e 0+e],[0 1 1 1-e 1-e 0+e],c3);plot([0 1 1 0 0],[0 0 1 1 0]);disp('Weights');
  "IW{1,1}(156,:)'" : Constant  Value=[0.90896921800109231615039107055054046213626861572265625;1.521414461285117258881882662535645067691802978515625;-2.12261668531512892599266706383787095546722412109375;-2.0157086381538480424069348373450338840484619140625;-2.114229456542515261929793268791399896144866943359375]
      mask Display: e = 0.06;c1 = [120 150 230]/255;c2 = ([120 150 230]+0)/383;c3 = ([120 150 230]+128)/383;patch([0 1 1 0],[0 0 1 1],c1);patch([0 1 1 1-e 1-e 0+e],[0 0 1 1-e 0+e 0+e],c2);patch([0 0 1 1-e 0+e 0+e],[0 1 1 1-e 1-e 0+e],c3);plot([0 1 1 0 0],[0 0 1 1 0]);disp('Weights');
  "IW{1,1}(157,:)'" : Constant  Value=[-2.27453209879713913466048325062729418277740478515625;1.980697714506566509129470432526431977748870849609375;1.5500381972804964103573865941143594682216644287109375;2.01071406883075542992855844204314053058624267578125;0.7645495199915106621091354099917225539684295654296875]
      mask Display: e = 0.06;c1 = [120 150 230]/255;c2 = ([120 150 230]+0)/383;c3 = ([120 150 230]+128)/383;patch([0 1 1 0],[0 0 1 1],c1);patch([0 1 1 1-e 1-e 0+e],[0 0 1 1-e 0+e 0+e],c2);patch([0 0 1 1-e 0+e 0+e],[0 1 1 1-e 1-e 0+e],c3);plot([0 1 1 0 0],[0 0 1 1 0]);disp('Weights');
  "IW{1,1}(158,:)'" : Constant  Value=[2.042173965459927575949450329062528908252716064453125;1.251131132979668603155687378603033721446990966796875;1.7193116995917867573240300771431066095829010009765625;1.8631750008109702054781564584118314087390899658203125;1.2514697277170674372115399819449521601200103759765625]
      mask Display: e = 0.06;c1 = [120 150 230]/255;c2 = ([120 150 230]+0)/383;c3 = ([120 150 230]+128)/383;patch([0 1 1 0],[0 0 1 1],c1);patch([0 1 1 1-e 1-e 0+e],[0 0 1 1-e 0+e 0+e],c2);patch([0 0 1 1-e 0+e 0+e],[0 1 1 1-e 1-e 0+e],c3);plot([0 1 1 0 0],[0 0 1 1 0]);disp('Weights');
  "IW{1,1}(159,:)'" : Constant  Value=[-2.246285807182043736673904277267865836620330810546875;0.67604436506970377873670940971351228654384613037109375;-1.037261693593758860032494339975528419017791748046875;2.12195207516085648791204221197403967380523681640625;2.231684040919219125242989321122877299785614013671875]
      mask Display: e = 0.06;c1 = [120 150 230]/255;c2 = ([120 150 230]+0)/383;c3 = ([120 150 230]+128)/383;patch([0 1 1 0],[0 0 1 1],c1);patch([0 1 1 1-e 1-e 0+e],[0 0 1 1-e 0+e 0+e],c2);patch([0 0 1 1-e 0+e 0+e],[0 1 1 1-e 1-e 0+e],c3);plot([0 1 1 0 0],[0 0 1 1 0]);disp('Weights');
  "IW{1,1}(16,:)'" : Constant  Value=[0.70307092125819503625194784035556949675083160400390625;-1.11838206583602328691995353437960147857666015625;1.9284812275137286352588716908940114080905914306640625;2.540461098112837046159029341652058064937591552734375;2.3831926991200536036785706528462469577789306640625]
      mask Display: e = 0.06;c1 = [120 150 230]/255;c2 = ([120 150 230]+0)/383;c3 = ([120 150 230]+128)/383;patch([0 1 1 0],[0 0 1 1],c1);patch([0 1 1 1-e 1-e 0+e],[0 0 1 1-e 0+e 0+e],c2);patch([0 0 1 1-e 0+e 0+e],[0 1 1 1-e 1-e 0+e],c3);plot([0 1 1 0 0],[0 0 1 1 0]);disp('Weights');
  "IW{1,1}(160,:)'" : Constant  Value=[0.568535730964966123934800634742714464664459228515625;-2.243418958996732381905303554958663880825042724609375;2.454589693524293014803561163716949522495269775390625;1.91763229916318334034031067858450114727020263671875;-1.264684694549553345410686233663000166416168212890625]
      mask Display: e = 0.06;c1 = [120 150 230]/255;c2 = ([120 150 230]+0)/383;c3 = ([120 150 230]+128)/383;patch([0 1 1 0],[0 0 1 1],c1);patch([0 1 1 1-e 1-e 0+e],[0 0 1 1-e 0+e 0+e],c2);patch([0 0 1 1-e 0+e 0+e],[0 1 1 1-e 1-e 0+e],c3);plot([0 1 1 0 0],[0 0 1 1 0]);disp('Weights');
  "IW{1,1}(161,:)'" : Constant  Value=[2.017470205717053932659155179862864315509796142578125;-1.6353649522575981478667017654515802860260009765625;-0.95199546045907867952706737924017943441867828369140625;-2.560247395078164789339325579931028187274932861328125;-1.039229304318536772910874788067303597927093505859375]
      mask Display: e = 0.06;c1 = [120 150 230]/255;c2 = ([120 150 230]+0)/383;c3 = ([120 150 230]+128)/383;patch([0 1 1 0],[0 0 1 1],c1);patch([0 1 1 1-e 1-e 0+e],[0 0 1 1-e 0+e 0+e],c2);patch([0 0 1 1-e 0+e 0+e],[0 1 1 1-e 1-e 0+e],c3);plot([0 1 1 0 0],[0 0 1 1 0]);disp('Weights');
  "IW{1,1}(162,:)'" : Constant  Value=[2.190025667923113150692415729281492531299591064453125;2.479805378252224468127451473264954984188079833984375;-2.091931919054101474131357463193126022815704345703125;0.95479866954810288515176353030255995690822601318359375;-1.4107430045534663509698702910100109875202178955078125]
      mask Display: e = 0.06;c1 = [120 150 230]/255;c2 = ([120 150 230]+0)/383;c3 = ([120 150 230]+128)/383;patch([0 1 1 0],[0 0 1 1],c1);patch([0 1 1 1-e 1-e 0+e],[0 0 1 1-e 0+e 0+e],c2);patch([0 0 1 1-e 0+e 0+e],[0 1 1 1-e 1-e 0+e],c3);plot([0 1 1 0 0],[0 0 1 1 0]);disp('Weights');
  "IW{1,1}(163,:)'" : Constant  Value=[-0.14623563479739498660592289525084197521209716796875;-1.601841898502979422147518562269397079944610595703125;-2.186726825887854719354663757258094847202301025390625;-3.0684111221650933742921552038751542568206787109375;-1.027690531269798146496441404451616108417510986328125]
      mask Display: e = 0.06;c1 = [120 150 230]/255;c2 = ([120 150 230]+0)/383;c3 = ([120 150 230]+128)/383;patch([0 1 1 0],[0 0 1 1],c1);patch([0 1 1 1-e 1-e 0+e],[0 0 1 1-e 0+e 0+e],c2);patch([0 0 1 1-e 0+e 0+e],[0 1 1 1-e 1-e 0+e],c3);plot([0 1 1 0 0],[0 0 1 1 0]);disp('Weights');
  "IW{1,1}(164,:)'" : Constant  Value=[2.81926140685358195270282521960325539112091064453125;1.8968218042178601745462174221756868064403533935546875;0.69981683630699065279401338557363487780094146728515625;1.48892900465697852752100516227073967456817626953125;-1.6141609780344337021773526430479250848293304443359375]
      mask Display: e = 0.06;c1 = [120 150 230]/255;c2 = ([120 150 230]+0)/383;c3 = ([120 150 230]+128)/383;patch([0 1 1 0],[0 0 1 1],c1);patch([0 1 1 1-e 1-e 0+e],[0 0 1 1-e 0+e 0+e],c2);patch([0 0 1 1-e 0+e 0+e],[0 1 1 1-e 1-e 0+e],c3);plot([0 1 1 0 0],[0 0 1 1 0]);disp('Weights');
  "IW{1,1}(165,:)'" : Constant  Value=[2.443735361193473121232955236337147653102874755859375;1.7518037300804232270223792511387728154659271240234375;0.455088586550156992682758527735131792724132537841796875;2.133777875209201813078152554226107895374298095703125;-1.0667877759774928581038011543569155037403106689453125]
      mask Display: e = 0.06;c1 = [120 150 230]/255;c2 = ([120 150 230]+0)/383;c3 = ([120 150 230]+128)/383;patch([0 1 1 0],[0 0 1 1],c1);patch([0 1 1 1-e 1-e 0+e],[0 0 1 1-e 0+e 0+e],c2);patch([0 0 1 1-e 0+e 0+e],[0 1 1 1-e 1-e 0+e],c3);plot([0 1 1 0 0],[0 0 1 1 0]);disp('Weights');
  "IW{1,1}(166,:)'" : Constant  Value=[2.2624370744491528739672503434121608734130859375;-1.75984165924330238084394295583479106426239013671875;0.1290701423047564133650411122289369814097881317138671875;-0.77663288093571491987887611685437150299549102783203125;2.62002283913343969601328353746794164180755615234375]
      mask Display: e = 0.06;c1 = [120 150 230]/255;c2 = ([120 150 230]+0)/383;c3 = ([120 150 230]+128)/383;patch([0 1 1 0],[0 0 1 1],c1);patch([0 1 1 1-e 1-e 0+e],[0 0 1 1-e 0+e 0+e],c2);patch([0 0 1 1-e 0+e 0+e],[0 1 1 1-e 1-e 0+e],c3);plot([0 1 1 0 0],[0 0 1 1 0]);disp('Weights');
  "IW{1,1}(167,:)'" : Constant  Value=[-2.592799588449730574524210169329307973384857177734375;0.3424696119850481057511615290422923862934112548828125;-1.756694573741546694378712345496751368045806884765625;2.508899249358852667768360333866439759731292724609375;-1.006190725330006419113715310231782495975494384765625]
      mask Display: e = 0.06;c1 = [120 150 230]/255;c2 = ([120 150 230]+0)/383;c3 = ([120 150 230]+128)/383;patch([0 1 1 0],[0 0 1 1],c1);patch([0 1 1 1-e 1-e 0+e],[0 0 1 1-e 0+e 0+e],c2);patch([0 0 1 1-e 0+e 0+e],[0 1 1 1-e 1-e 0+e],c3);plot([0 1 1 0 0],[0 0 1 1 0]);disp('Weights');
  "IW{1,1}(168,:)'" : Constant  Value=[-0.293214065518589694914197707475977949798107147216796875;-2.22734370771988121617823708220385015010833740234375;-2.612637333298014841176382105913944542407989501953125;-2.802869914344900958980133509612642228603363037109375;-1.5103294522214449902008936987840570509433746337890625]
      mask Display: e = 0.06;c1 = [120 150 230]/255;c2 = ([120 150 230]+0)/383;c3 = ([120 150 230]+128)/383;patch([0 1 1 0],[0 0 1 1],c1);patch([0 1 1 1-e 1-e 0+e],[0 0 1 1-e 0+e 0+e],c2);patch([0 0 1 1-e 0+e 0+e],[0 1 1 1-e 1-e 0+e],c3);plot([0 1 1 0 0],[0 0 1 1 0]);disp('Weights');
  "IW{1,1}(169,:)'" : Constant  Value=[1.8564804618053727391924212497542612254619598388671875;-2.798469931303891211626932999934069812297821044921875;-1.9409161029943475806902597469161264598369598388671875;0.244646194754816803662578195144305936992168426513671875;0.700621787543627139172031093039549887180328369140625]
      mask Display: e = 0.06;c1 = [120 150 230]/255;c2 = ([120 150 230]+0)/383;c3 = ([120 150 230]+128)/383;patch([0 1 1 0],[0 0 1 1],c1);patch([0 1 1 1-e 1-e 0+e],[0 0 1 1-e 0+e 0+e],c2);patch([0 0 1 1-e 0+e 0+e],[0 1 1 1-e 1-e 0+e],c3);plot([0 1 1 0 0],[0 0 1 1 0]);disp('Weights');
  "IW{1,1}(17,:)'" : Constant  Value=[0.96878320013974084101704420390888117253780364990234375;3.575054908951494692104233763529919087886810302734375;0.74875768147466892354913170493091456592082977294921875;0.7877282773014051553417402828927151858806610107421875;2.732656957839727507320048971450887620449066162109375]
      mask Display: e = 0.06;c1 = [120 150 230]/255;c2 = ([120 150 230]+0)/383;c3 = ([120 150 230]+128)/383;patch([0 1 1 0],[0 0 1 1],c1);patch([0 1 1 1-e 1-e 0+e],[0 0 1 1-e 0+e 0+e],c2);patch([0 0 1 1-e 0+e 0+e],[0 1 1 1-e 1-e 0+e],c3);plot([0 1 1 0 0],[0 0 1 1 0]);disp('Weights');
  "IW{1,1}(170,:)'" : Constant  Value=[-1.452444187212368120754035771824419498443603515625;1.846039604050389915101959559251554310321807861328125;-1.6076475106426311167950871094944886863231658935546875;1.0467954397004006761306982298265211284160614013671875;-2.10716632463906794470176464528776705265045166015625]
      mask Display: e = 0.06;c1 = [120 150 230]/255;c2 = ([120 150 230]+0)/383;c3 = ([120 150 230]+128)/383;patch([0 1 1 0],[0 0 1 1],c1);patch([0 1 1 1-e 1-e 0+e],[0 0 1 1-e 0+e 0+e],c2);patch([0 0 1 1-e 0+e 0+e],[0 1 1 1-e 1-e 0+e],c3);plot([0 1 1 0 0],[0 0 1 1 0]);disp('Weights');
  "IW{1,1}(171,:)'" : Constant  Value=[1.4582176874219181517133847592049278318881988525390625;-2.844021226224720866326833856874145567417144775390625;1.239803346185132770784775857464410364627838134765625;1.2644265035155430876301352327573113143444061279296875;-1.75557744938285420488455201848410069942474365234375]
      mask Display: e = 0.06;c1 = [120 150 230]/255;c2 = ([120 150 230]+0)/383;c3 = ([120 150 230]+128)/383;patch([0 1 1 0],[0 0 1 1],c1);patch([0 1 1 1-e 1-e 0+e],[0 0 1 1-e 0+e 0+e],c2);patch([0 0 1 1-e 0+e 0+e],[0 1 1 1-e 1-e 0+e],c3);plot([0 1 1 0 0],[0 0 1 1 0]);disp('Weights');
  "IW{1,1}(172,:)'" : Constant  Value=[-0.5849934776255611978967863251455128192901611328125;-1.4301923286554216740995570944505743682384490966796875;-0.54021101946546978833652019602595828473567962646484375;-2.41865734768328533021986004314385354518890380859375;2.86146285610000017385345927323214709758758544921875]
      mask Display: e = 0.06;c1 = [120 150 230]/255;c2 = ([120 150 230]+0)/383;c3 = ([120 150 230]+128)/383;patch([0 1 1 0],[0 0 1 1],c1);patch([0 1 1 1-e 1-e 0+e],[0 0 1 1-e 0+e 0+e],c2);patch([0 0 1 1-e 0+e 0+e],[0 1 1 1-e 1-e 0+e],c3);plot([0 1 1 0 0],[0 0 1 1 0]);disp('Weights');
  "IW{1,1}(173,:)'" : Constant  Value=[0.8058300373850073583525954745709896087646484375;-1.7292127953551614805149938547401688992977142333984375;-2.731114093896747530010316040716134011745452880859375;-1.6082508979304079854699693896691314876079559326171875;0.7149818569233168386034549257601611316204071044921875]
      mask Display: e = 0.06;c1 = [120 150 230]/255;c2 = ([120 150 230]+0)/383;c3 = ([120 150 230]+128)/383;patch([0 1 1 0],[0 0 1 1],c1);patch([0 1 1 1-e 1-e 0+e],[0 0 1 1-e 0+e 0+e],c2);patch([0 0 1 1-e 0+e 0+e],[0 1 1 1-e 1-e 0+e],c3);plot([0 1 1 0 0],[0 0 1 1 0]);disp('Weights');
  "IW{1,1}(174,:)'" : Constant  Value=[-1.3180991206651049285625276752398349344730377197265625;-1.6401077051685690744164958232431672513484954833984375;1.314522687280038848456342748249880969524383544921875;2.60563835525004083848443769966252148151397705078125;-1.6926473763750171652731069116271100938320159912109375]
      mask Display: e = 0.06;c1 = [120 150 230]/255;c2 = ([120 150 230]+0)/383;c3 = ([120 150 230]+128)/383;patch([0 1 1 0],[0 0 1 1],c1);patch([0 1 1 1-e 1-e 0+e],[0 0 1 1-e 0+e 0+e],c2);patch([0 0 1 1-e 0+e 0+e],[0 1 1 1-e 1-e 0+e],c3);plot([0 1 1 0 0],[0 0 1 1 0]);disp('Weights');
  "IW{1,1}(175,:)'" : Constant  Value=[-2.47413302220083775040393447852693498134613037109375;1.0497156572083792269722835044376552104949951171875;-1.9321277420941342928273343204637058079242706298828125;0.76178390965919129396155540234758518636226654052734375;2.1518990473653243356011444120667874813079833984375]
      mask Display: e = 0.06;c1 = [120 150 230]/255;c2 = ([120 150 230]+0)/383;c3 = ([120 150 230]+128)/383;patch([0 1 1 0],[0 0 1 1],c1);patch([0 1 1 1-e 1-e 0+e],[0 0 1 1-e 0+e 0+e],c2);patch([0 0 1 1-e 0+e 0+e],[0 1 1 1-e 1-e 0+e],c3);plot([0 1 1 0 0],[0 0 1 1 0]);disp('Weights');
  "IW{1,1}(176,:)'" : Constant  Value=[-1.17705988034265107700093722087331116199493408203125;2.4285492769125962553289355128072202205657958984375;1.77946090184522365262864695978350937366485595703125;-2.37427990957022938545151191647164523601531982421875;-0.444934626423984458387650420263526029884815216064453125]
      mask Display: e = 0.06;c1 = [120 150 230]/255;c2 = ([120 150 230]+0)/383;c3 = ([120 150 230]+128)/383;patch([0 1 1 0],[0 0 1 1],c1);patch([0 1 1 1-e 1-e 0+e],[0 0 1 1-e 0+e 0+e],c2);patch([0 0 1 1-e 0+e 0+e],[0 1 1 1-e 1-e 0+e],c3);plot([0 1 1 0 0],[0 0 1 1 0]);disp('Weights');
  "IW{1,1}(177,:)'" : Constant  Value=[2.58317448302465901832647432456724345684051513671875;-2.991385348785570830187907631625421345233917236328125;0.10151073912681267408242291594433481805026531219482421875;0.80654230351143707533623228300712071359157562255859375;0.294132477570214601048093072677147574722766876220703125]
      mask Display: e = 0.06;c1 = [120 150 230]/255;c2 = ([120 150 230]+0)/383;c3 = ([120 150 230]+128)/383;patch([0 1 1 0],[0 0 1 1],c1);patch([0 1 1 1-e 1-e 0+e],[0 0 1 1-e 0+e 0+e],c2);patch([0 0 1 1-e 0+e 0+e],[0 1 1 1-e 1-e 0+e],c3);plot([0 1 1 0 0],[0 0 1 1 0]);disp('Weights');
  "IW{1,1}(178,:)'" : Constant  Value=[-0.299875001185044454121708668026258237659931182861328125;2.47763601766333874110159740666858851909637451171875;0.4793837087674945873772003324120305478572845458984375;-3.118776648021637232233160830219276249408721923828125;0.279657589235684789219504864377086050808429718017578125]
      mask Display: e = 0.06;c1 = [120 150 230]/255;c2 = ([120 150 230]+0)/383;c3 = ([120 150 230]+128)/383;patch([0 1 1 0],[0 0 1 1],c1);patch([0 1 1 1-e 1-e 0+e],[0 0 1 1-e 0+e 0+e],c2);patch([0 0 1 1-e 0+e 0+e],[0 1 1 1-e 1-e 0+e],c3);plot([0 1 1 0 0],[0 0 1 1 0]);disp('Weights');
  "IW{1,1}(179,:)'" : Constant  Value=[-1.5369244221710649522805169908679090440273284912109375;1.7856846304983944317967825554660521447658538818359375;-1.9393030779207769409566708418424241244792938232421875;1.563666995682127858202647985308431088924407958984375;-2.143855156756108382154479841119609773159027099609375]
      mask Display: e = 0.06;c1 = [120 150 230]/255;c2 = ([120 150 230]+0)/383;c3 = ([120 150 230]+128)/383;patch([0 1 1 0],[0 0 1 1],c1);patch([0 1 1 1-e 1-e 0+e],[0 0 1 1-e 0+e 0+e],c2);patch([0 0 1 1-e 0+e 0+e],[0 1 1 1-e 1-e 0+e],c3);plot([0 1 1 0 0],[0 0 1 1 0]);disp('Weights');
  "IW{1,1}(18,:)'" : Constant  Value=[2.6516149785083928946960440953262150287628173828125;-2.395307557333805181798425110173411667346954345703125;0.347227172789360383209356086808838881552219390869140625;1.5731788054961228784378590717096813023090362548828125;-0.96809556871637492125870494419359602034091949462890625]
      mask Display: e = 0.06;c1 = [120 150 230]/255;c2 = ([120 150 230]+0)/383;c3 = ([120 150 230]+128)/383;patch([0 1 1 0],[0 0 1 1],c1);patch([0 1 1 1-e 1-e 0+e],[0 0 1 1-e 0+e 0+e],c2);patch([0 0 1 1-e 0+e 0+e],[0 1 1 1-e 1-e 0+e],c3);plot([0 1 1 0 0],[0 0 1 1 0]);disp('Weights');
  "IW{1,1}(180,:)'" : Constant  Value=[1.2342689464412590627517829489079304039478302001953125;1.917414011047894550898718080134131014347076416015625;1.4310857136857231264315259977593086659908294677734375;1.8609147524433400366916657731053419411182403564453125;-2.43786449753017908648189404630102217197418212890625]
      mask Display: e = 0.06;c1 = [120 150 230]/255;c2 = ([120 150 230]+0)/383;c3 = ([120 150 230]+128)/383;patch([0 1 1 0],[0 0 1 1],c1);patch([0 1 1 1-e 1-e 0+e],[0 0 1 1-e 0+e 0+e],c2);patch([0 0 1 1-e 0+e 0+e],[0 1 1 1-e 1-e 0+e],c3);plot([0 1 1 0 0],[0 0 1 1 0]);disp('Weights');
  "IW{1,1}(181,:)'" : Constant  Value=[1.85020680363616651931124579277820885181427001953125;3.37384809595060186637738297577016055583953857421875;0.385305837709988441286412808040040545165538787841796875;-1.1291494759279332438239862312912009656429290771484375;-0.1218717150861522158233896107049076817929744720458984375]
      mask Display: e = 0.06;c1 = [120 150 230]/255;c2 = ([120 150 230]+0)/383;c3 = ([120 150 230]+128)/383;patch([0 1 1 0],[0 0 1 1],c1);patch([0 1 1 1-e 1-e 0+e],[0 0 1 1-e 0+e 0+e],c2);patch([0 0 1 1-e 0+e 0+e],[0 1 1 1-e 1-e 0+e],c3);plot([0 1 1 0 0],[0 0 1 1 0]);disp('Weights');
  "IW{1,1}(182,:)'" : Constant  Value=[-2.193948494609151200762653388665057718753814697265625;-1.783068311932206828629432493471540510654449462890625;-0.002597345689584375748315547838274142122827470302581787109375;-1.575135793987811894112383015453815460205078125;-1.8159210420558784537803376224474050104618072509765625]
      mask Display: e = 0.06;c1 = [120 150 230]/255;c2 = ([120 150 230]+0)/383;c3 = ([120 150 230]+128)/383;patch([0 1 1 0],[0 0 1 1],c1);patch([0 1 1 1-e 1-e 0+e],[0 0 1 1-e 0+e 0+e],c2);patch([0 0 1 1-e 0+e 0+e],[0 1 1 1-e 1-e 0+e],c3);plot([0 1 1 0 0],[0 0 1 1 0]);disp('Weights');
  "IW{1,1}(183,:)'" : Constant  Value=[3.1277135066373791261185033363290131092071533203125;0.122618644589532532762632399681024253368377685546875;-0.843147079701937141038570189266465604305267333984375;2.460350377377134467593577937805093824863433837890625;-0.3326729889667741080216956106596626341342926025390625]
      mask Display: e = 0.06;c1 = [120 150 230]/255;c2 = ([120 150 230]+0)/383;c3 = ([120 150 230]+128)/383;patch([0 1 1 0],[0 0 1 1],c1);patch([0 1 1 1-e 1-e 0+e],[0 0 1 1-e 0+e 0+e],c2);patch([0 0 1 1-e 0+e 0+e],[0 1 1 1-e 1-e 0+e],c3);plot([0 1 1 0 0],[0 0 1 1 0]);disp('Weights');
  "IW{1,1}(184,:)'" : Constant  Value=[1.886999909949029774480777632561512291431427001953125;1.7952810144961011129538519526249729096889495849609375;1.220532192287997919066810936783440411090850830078125;-1.6922187710335154786633893309044651687145233154296875;-0.0190598785924090512178263878695361199788749217987060546875]
      mask Display: e = 0.06;c1 = [120 150 230]/255;c2 = ([120 150 230]+0)/383;c3 = ([120 150 230]+128)/383;patch([0 1 1 0],[0 0 1 1],c1);patch([0 1 1 1-e 1-e 0+e],[0 0 1 1-e 0+e 0+e],c2);patch([0 0 1 1-e 0+e 0+e],[0 1 1 1-e 1-e 0+e],c3);plot([0 1 1 0 0],[0 0 1 1 0]);disp('Weights');
  "IW{1,1}(185,:)'" : Constant  Value=[-1.7669934821822510517819182496168650686740875244140625;0.87072623929937897901965015989844687283039093017578125;-3.6870698475729835053016358870081603527069091796875;-1.737953750987852874487771259737201035022735595703125;1.40285917273684379580345193971879780292510986328125]
      mask Display: e = 0.06;c1 = [120 150 230]/255;c2 = ([120 150 230]+0)/383;c3 = ([120 150 230]+128)/383;patch([0 1 1 0],[0 0 1 1],c1);patch([0 1 1 1-e 1-e 0+e],[0 0 1 1-e 0+e 0+e],c2);patch([0 0 1 1-e 0+e 0+e],[0 1 1 1-e 1-e 0+e],c3);plot([0 1 1 0 0],[0 0 1 1 0]);disp('Weights');
  "IW{1,1}(186,:)'" : Constant  Value=[0.9243733457756964089213624902185983955860137939453125;2.476979895106173668040128177381120622158050537109375;0.523267800844552599670578274526633322238922119140625;-1.626098236523855877777577916276641190052032470703125;-2.53199114147551807008085233974270522594451904296875]
      mask Display: e = 0.06;c1 = [120 150 230]/255;c2 = ([120 150 230]+0)/383;c3 = ([120 150 230]+128)/383;patch([0 1 1 0],[0 0 1 1],c1);patch([0 1 1 1-e 1-e 0+e],[0 0 1 1-e 0+e 0+e],c2);patch([0 0 1 1-e 0+e 0+e],[0 1 1 1-e 1-e 0+e],c3);plot([0 1 1 0 0],[0 0 1 1 0]);disp('Weights');
  "IW{1,1}(187,:)'" : Constant  Value=[-1.0206646726649761802718785475008189678192138671875;2.380127235383919792610640797647647559642791748046875;1.9265595357553080280155199943692423403263092041015625;-2.211774674259129103148779904586263000965118408203125;1.129042730976129949027608745382167398929595947265625]
      mask Display: e = 0.06;c1 = [120 150 230]/255;c2 = ([120 150 230]+0)/383;c3 = ([120 150 230]+128)/383;patch([0 1 1 0],[0 0 1 1],c1);patch([0 1 1 1-e 1-e 0+e],[0 0 1 1-e 0+e 0+e],c2);patch([0 0 1 1-e 0+e 0+e],[0 1 1 1-e 1-e 0+e],c3);plot([0 1 1 0 0],[0 0 1 1 0]);disp('Weights');
  "IW{1,1}(188,:)'" : Constant  Value=[2.192787449399648647130334211396984755992889404296875;2.562871169049651509652676395489834249019622802734375;-0.21316828314868441207607929754885844886302947998046875;0.348241384771730999592165289868717081844806671142578125;-1.874270337859898827304050428210757672786712646484375]
      mask Display: e = 0.06;c1 = [120 150 230]/255;c2 = ([120 150 230]+0)/383;c3 = ([120 150 230]+128)/383;patch([0 1 1 0],[0 0 1 1],c1);patch([0 1 1 1-e 1-e 0+e],[0 0 1 1-e 0+e 0+e],c2);patch([0 0 1 1-e 0+e 0+e],[0 1 1 1-e 1-e 0+e],c3);plot([0 1 1 0 0],[0 0 1 1 0]);disp('Weights');
  "IW{1,1}(189,:)'" : Constant  Value=[-1.59901735379332965436560698435641825199127197265625;-3.35080036925182067619743975228630006313323974609375;0.99101490701186312204384876167750917375087738037109375;-0.80076196502289376244476670763106085360050201416015625;0.64130668830976322869474870458361692726612091064453125]
      mask Display: e = 0.06;c1 = [120 150 230]/255;c2 = ([120 150 230]+0)/383;c3 = ([120 150 230]+128)/383;patch([0 1 1 0],[0 0 1 1],c1);patch([0 1 1 1-e 1-e 0+e],[0 0 1 1-e 0+e 0+e],c2);patch([0 0 1 1-e 0+e 0+e],[0 1 1 1-e 1-e 0+e],c3);plot([0 1 1 0 0],[0 0 1 1 0]);disp('Weights');
  "IW{1,1}(19,:)'" : Constant  Value=[1.81930411712207185104261952801607549190521240234375;1.8323061304384451464244421003968454897403717041015625;1.01534180010217855993914781720377504825592041015625;-2.92954308027117971136021878919564187526702880859375;-0.1094649023711161961447402291014441289007663726806640625]
      mask Display: e = 0.06;c1 = [120 150 230]/255;c2 = ([120 150 230]+0)/383;c3 = ([120 150 230]+128)/383;patch([0 1 1 0],[0 0 1 1],c1);patch([0 1 1 1-e 1-e 0+e],[0 0 1 1-e 0+e 0+e],c2);patch([0 0 1 1-e 0+e 0+e],[0 1 1 1-e 1-e 0+e],c3);plot([0 1 1 0 0],[0 0 1 1 0]);disp('Weights');
  "IW{1,1}(190,:)'" : Constant  Value=[-2.745304359304764574289947631768882274627685546875;-0.44505311494080768142111992347054183483123779296875;-1.6109549685540469621258807819685898721218109130859375;2.1475819764538588430013987817801535129547119140625;1.0084406323412864470157046525855548679828643798828125]
      mask Display: e = 0.06;c1 = [120 150 230]/255;c2 = ([120 150 230]+0)/383;c3 = ([120 150 230]+128)/383;patch([0 1 1 0],[0 0 1 1],c1);patch([0 1 1 1-e 1-e 0+e],[0 0 1 1-e 0+e 0+e],c2);patch([0 0 1 1-e 0+e 0+e],[0 1 1 1-e 1-e 0+e],c3);plot([0 1 1 0 0],[0 0 1 1 0]);disp('Weights');
  "IW{1,1}(191,:)'" : Constant  Value=[2.357111484098833198430611446383409202098846435546875;-1.77040646136406198962731650681234896183013916015625;0.9705837642731831582665336100035347044467926025390625;-0.12499557855189911970139604591167881153523921966552734375;2.5188091332544022549200235516764223575592041015625]
      mask Display: e = 0.06;c1 = [120 150 230]/255;c2 = ([120 150 230]+0)/383;c3 = ([120 150 230]+128)/383;patch([0 1 1 0],[0 0 1 1],c1);patch([0 1 1 1-e 1-e 0+e],[0 0 1 1-e 0+e 0+e],c2);patch([0 0 1 1-e 0+e 0+e],[0 1 1 1-e 1-e 0+e],c3);plot([0 1 1 0 0],[0 0 1 1 0]);disp('Weights');
  "IW{1,1}(192,:)'" : Constant  Value=[0.09531393594501703925292446228922926820814609527587890625;-2.712852625150846019863593028276227414608001708984375;-1.62593078161754345245526565122418105602264404296875;-0.99892102155383033501578893265104852616786956787109375;-3.460434611194439735726291473838500678539276123046875]
      mask Display: e = 0.06;c1 = [120 150 230]/255;c2 = ([120 150 230]+0)/383;c3 = ([120 150 230]+128)/383;patch([0 1 1 0],[0 0 1 1],c1);patch([0 1 1 1-e 1-e 0+e],[0 0 1 1-e 0+e 0+e],c2);patch([0 0 1 1-e 0+e 0+e],[0 1 1 1-e 1-e 0+e],c3);plot([0 1 1 0 0],[0 0 1 1 0]);disp('Weights');
  "IW{1,1}(193,:)'" : Constant  Value=[0.8268049491121656213721280437312088906764984130859375;-1.9613556668727143428299086735933087766170501708984375;1.610553374924624137065620743669569492340087890625;-2.3558625279985800915483196149580180644989013671875;1.9085968743368615374578212140477262437343597412109375]
      mask Display: e = 0.06;c1 = [120 150 230]/255;c2 = ([120 150 230]+0)/383;c3 = ([120 150 230]+128)/383;patch([0 1 1 0],[0 0 1 1],c1);patch([0 1 1 1-e 1-e 0+e],[0 0 1 1-e 0+e 0+e],c2);patch([0 0 1 1-e 0+e 0+e],[0 1 1 1-e 1-e 0+e],c3);plot([0 1 1 0 0],[0 0 1 1 0]);disp('Weights');
  "IW{1,1}(194,:)'" : Constant  Value=[2.43053042006148078968408299260772764682769775390625;1.4088852418326698323625123521196655929088592529296875;1.72416612787749645718804458738304674625396728515625;-1.4383908511051892720189471219782717525959014892578125;-0.9205332244073718417354257326223887503147125244140625]
      mask Display: e = 0.06;c1 = [120 150 230]/255;c2 = ([120 150 230]+0)/383;c3 = ([120 150 230]+128)/383;patch([0 1 1 0],[0 0 1 1],c1);patch([0 1 1 1-e 1-e 0+e],[0 0 1 1-e 0+e 0+e],c2);patch([0 0 1 1-e 0+e 0+e],[0 1 1 1-e 1-e 0+e],c3);plot([0 1 1 0 0],[0 0 1 1 0]);disp('Weights');
  "IW{1,1}(195,:)'" : Constant  Value=[-1.4980763054289811808672538973041810095310211181640625;0.200157863137303049239079655308159999549388885498046875;3.641638346741054466093601149623282253742218017578125;0.35267362926543199819207075051963329315185546875;-0.80414425230768260544067516093491576611995697021484375]
      mask Display: e = 0.06;c1 = [120 150 230]/255;c2 = ([120 150 230]+0)/383;c3 = ([120 150 230]+128)/383;patch([0 1 1 0],[0 0 1 1],c1);patch([0 1 1 1-e 1-e 0+e],[0 0 1 1-e 0+e 0+e],c2);patch([0 0 1 1-e 0+e 0+e],[0 1 1 1-e 1-e 0+e],c3);plot([0 1 1 0 0],[0 0 1 1 0]);disp('Weights');
  "IW{1,1}(196,:)'" : Constant  Value=[-2.782874945961119284021378916804678738117218017578125;2.617099569382550061646952599403448402881622314453125;-0.486292376310839935538155032190843485295772552490234375;-0.71322157392192064850888755245250649750232696533203125;-1.24243076390949713783129482180811464786529541015625]
      mask Display: e = 0.06;c1 = [120 150 230]/255;c2 = ([120 150 230]+0)/383;c3 = ([120 150 230]+128)/383;patch([0 1 1 0],[0 0 1 1],c1);patch([0 1 1 1-e 1-e 0+e],[0 0 1 1-e 0+e 0+e],c2);patch([0 0 1 1-e 0+e 0+e],[0 1 1 1-e 1-e 0+e],c3);plot([0 1 1 0 0],[0 0 1 1 0]);disp('Weights');
  "IW{1,1}(197,:)'" : Constant  Value=[1.495982681143153580904936461593024432659149169921875;2.52394169392909173410544099169783294200897216796875;0.3590289691583412601261215968406759202480316162109375;2.812326763905872883952952179242856800556182861328125;0.56401216322592462315554939777939580380916595458984375]
      mask Display: e = 0.06;c1 = [120 150 230]/255;c2 = ([120 150 230]+0)/383;c3 = ([120 150 230]+128)/383;patch([0 1 1 0],[0 0 1 1],c1);patch([0 1 1 1-e 1-e 0+e],[0 0 1 1-e 0+e 0+e],c2);patch([0 0 1 1-e 0+e 0+e],[0 1 1 1-e 1-e 0+e],c3);plot([0 1 1 0 0],[0 0 1 1 0]);disp('Weights');
  "IW{1,1}(198,:)'" : Constant  Value=[-1.6570208589384465280858194091706536710262298583984375;-1.441829704811109724715834090602584183216094970703125;0.2505220783689063868138191537582315504550933837890625;-3.435994174850966142997776842094026505947113037109375;-1.4573123674285517470394779593334533274173736572265625]
      mask Display: e = 0.06;c1 = [120 150 230]/255;c2 = ([120 150 230]+0)/383;c3 = ([120 150 230]+128)/383;patch([0 1 1 0],[0 0 1 1],c1);patch([0 1 1 1-e 1-e 0+e],[0 0 1 1-e 0+e 0+e],c2);patch([0 0 1 1-e 0+e 0+e],[0 1 1 1-e 1-e 0+e],c3);plot([0 1 1 0 0],[0 0 1 1 0]);disp('Weights');
  "IW{1,1}(199,:)'" : Constant  Value=[0.86670243903810983976399029415915720164775848388671875;-1.273935826385443892405646693077869713306427001953125;3.45557163997982907943651298410259187221527099609375;-0.55308842643264377603173898023669607937335968017578125;-1.3261050276598351782553208977333270013332366943359375]
      mask Display: e = 0.06;c1 = [120 150 230]/255;c2 = ([120 150 230]+0)/383;c3 = ([120 150 230]+128)/383;patch([0 1 1 0],[0 0 1 1],c1);patch([0 1 1 1-e 1-e 0+e],[0 0 1 1-e 0+e 0+e],c2);patch([0 0 1 1-e 0+e 0+e],[0 1 1 1-e 1-e 0+e],c3);plot([0 1 1 0 0],[0 0 1 1 0]);disp('Weights');
  "IW{1,1}(2,:)'" : Constant  Value=[2.417863521539576954211270276573486626148223876953125;-1.8245921379972198650420978083275258541107177734375;-1.2262822393714933877362227576668374240398406982421875;2.382655496602698708130674276617355644702911376953125;0.240038433424933861370931253986782394349575042724609375]
      mask Display: e = 0.06;c1 = [120 150 230]/255;c2 = ([120 150 230]+0)/383;c3 = ([120 150 230]+128)/383;patch([0 1 1 0],[0 0 1 1],c1);patch([0 1 1 1-e 1-e 0+e],[0 0 1 1-e 0+e 0+e],c2);patch([0 0 1 1-e 0+e 0+e],[0 1 1 1-e 1-e 0+e],c3);plot([0 1 1 0 0],[0 0 1 1 0]);disp('Weights');
  "IW{1,1}(20,:)'" : Constant  Value=[-1.2034255380141509750302475367789156734943389892578125;-2.29410689297241265904858664725907146930694580078125;-2.595880546827816548471901114680804312229156494140625;-0.1605937643934215175445245904484181664884090423583984375;1.282167042531336509370021303766407072544097900390625]
      mask Display: e = 0.06;c1 = [120 150 230]/255;c2 = ([120 150 230]+0)/383;c3 = ([120 150 230]+128)/383;patch([0 1 1 0],[0 0 1 1],c1);patch([0 1 1 1-e 1-e 0+e],[0 0 1 1-e 0+e 0+e],c2);patch([0 0 1 1-e 0+e 0+e],[0 1 1 1-e 1-e 0+e],c3);plot([0 1 1 0 0],[0 0 1 1 0]);disp('Weights');
  "IW{1,1}(200,:)'" : Constant  Value=[-1.576379525580170248844069647020660340785980224609375;-1.17297605242612945630753529258072376251220703125;-2.627254814727257414830319248721934854984283447265625;0.262014730920779370659801088550011627376079559326171875;-0.66882454116583189840383738555829040706157684326171875]
      mask Display: e = 0.06;c1 = [120 150 230]/255;c2 = ([120 150 230]+0)/383;c3 = ([120 150 230]+128)/383;patch([0 1 1 0],[0 0 1 1],c1);patch([0 1 1 1-e 1-e 0+e],[0 0 1 1-e 0+e 0+e],c2);patch([0 0 1 1-e 0+e 0+e],[0 1 1 1-e 1-e 0+e],c3);plot([0 1 1 0 0],[0 0 1 1 0]);disp('Weights');
  "IW{1,1}(21,:)'" : Constant  Value=[-0.20447642278898781054152777869603596627712249755859375;-0.589150086715275467241781370830722153186798095703125;-2.12899917175329189689136910601519048213958740234375;-3.395160752993839903268735724850557744503021240234375;1.3784842417361959920896197218098677694797515869140625]
      mask Display: e = 0.06;c1 = [120 150 230]/255;c2 = ([120 150 230]+0)/383;c3 = ([120 150 230]+128)/383;patch([0 1 1 0],[0 0 1 1],c1);patch([0 1 1 1-e 1-e 0+e],[0 0 1 1-e 0+e 0+e],c2);patch([0 0 1 1-e 0+e 0+e],[0 1 1 1-e 1-e 0+e],c3);plot([0 1 1 0 0],[0 0 1 1 0]);disp('Weights');
  "IW{1,1}(22,:)'" : Constant  Value=[-2.196000843496789034503535731346346437931060791015625;2.978938650868370618951530559570528566837310791015625;0.91614750503152941885076643302454613149166107177734375;1.4873710866835343491487719802535139024257659912109375;-0.51833158494691689011091284555732272565364837646484375]
      mask Display: e = 0.06;c1 = [120 150 230]/255;c2 = ([120 150 230]+0)/383;c3 = ([120 150 230]+128)/383;patch([0 1 1 0],[0 0 1 1],c1);patch([0 1 1 1-e 1-e 0+e],[0 0 1 1-e 0+e 0+e],c2);patch([0 0 1 1-e 0+e 0+e],[0 1 1 1-e 1-e 0+e],c3);plot([0 1 1 0 0],[0 0 1 1 0]);disp('Weights');
  "IW{1,1}(23,:)'" : Constant  Value=[2.2799897682074448113098696921952068805694580078125;-1.3534850006306784475640370146720670163631439208984375;-1.8892745399485890711588353951810859143733978271484375;1.9954022977659047199949782225303351879119873046875;-1.3131409421604354204049514009966515004634857177734375]
      mask Display: e = 0.06;c1 = [120 150 230]/255;c2 = ([120 150 230]+0)/383;c3 = ([120 150 230]+128)/383;patch([0 1 1 0],[0 0 1 1],c1);patch([0 1 1 1-e 1-e 0+e],[0 0 1 1-e 0+e 0+e],c2);patch([0 0 1 1-e 0+e 0+e],[0 1 1 1-e 1-e 0+e],c3);plot([0 1 1 0 0],[0 0 1 1 0]);disp('Weights');
  "IW{1,1}(24,:)'" : Constant  Value=[-1.98688520159929371544649256975390017032623291015625;-2.1983336166313645065883974893949925899505615234375;1.3249530937911389028016628799377940595149993896484375;2.116839439329335714745639052125625312328338623046875;-1.159541783119327096329698179033584892749786376953125]
      mask Display: e = 0.06;c1 = [120 150 230]/255;c2 = ([120 150 230]+0)/383;c3 = ([120 150 230]+128)/383;patch([0 1 1 0],[0 0 1 1],c1);patch([0 1 1 1-e 1-e 0+e],[0 0 1 1-e 0+e 0+e],c2);patch([0 0 1 1-e 0+e 0+e],[0 1 1 1-e 1-e 0+e],c3);plot([0 1 1 0 0],[0 0 1 1 0]);disp('Weights');
  "IW{1,1}(25,:)'" : Constant  Value=[1.8497359820516148243285670105251483619213104248046875;0.5199152442557721798266356927342712879180908203125;-1.55493669861581640390113534522242844104766845703125;1.2784565641990448536802205126150511205196380615234375;-2.83882187278945696817800126154907047748565673828125]
      mask Display: e = 0.06;c1 = [120 150 230]/255;c2 = ([120 150 230]+0)/383;c3 = ([120 150 230]+128)/383;patch([0 1 1 0],[0 0 1 1],c1);patch([0 1 1 1-e 1-e 0+e],[0 0 1 1-e 0+e 0+e],c2);patch([0 0 1 1-e 0+e 0+e],[0 1 1 1-e 1-e 0+e],c3);plot([0 1 1 0 0],[0 0 1 1 0]);disp('Weights');
  "IW{1,1}(26,:)'" : Constant  Value=[1.98101968983187237682841441710479557514190673828125;-1.42731777774352419640990774496458470821380615234375;-2.921008736887971135587349635898135602474212646484375;1.2216942181757859398061327738105319440364837646484375;-0.342137769993370255416920144853065721690654754638671875]
      mask Display: e = 0.06;c1 = [120 150 230]/255;c2 = ([120 150 230]+0)/383;c3 = ([120 150 230]+128)/383;patch([0 1 1 0],[0 0 1 1],c1);patch([0 1 1 1-e 1-e 0+e],[0 0 1 1-e 0+e 0+e],c2);patch([0 0 1 1-e 0+e 0+e],[0 1 1 1-e 1-e 0+e],c3);plot([0 1 1 0 0],[0 0 1 1 0]);disp('Weights');
  "IW{1,1}(27,:)'" : Constant  Value=[1.6163209299549148312280522077344357967376708984375;-1.9625434102941710090561855395208112895488739013671875;-1.07178098500552732019741597468964755535125732421875;2.149299883720892534455515487934462726116180419921875;-1.8274299915153775497600463495473377406597137451171875]
      mask Display: e = 0.06;c1 = [120 150 230]/255;c2 = ([120 150 230]+0)/383;c3 = ([120 150 230]+128)/383;patch([0 1 1 0],[0 0 1 1],c1);patch([0 1 1 1-e 1-e 0+e],[0 0 1 1-e 0+e 0+e],c2);patch([0 0 1 1-e 0+e 0+e],[0 1 1 1-e 1-e 0+e],c3);plot([0 1 1 0 0],[0 0 1 1 0]);disp('Weights');
  "IW{1,1}(28,:)'" : Constant  Value=[-2.326142558300211771182830489124171435832977294921875;2.828226226322665848300630386802367866039276123046875;0.7998673485353899881289407858275808393955230712890625;-0.46774984833188260058278729047742672264575958251953125;-1.45417748611337938058341023861430585384368896484375]
      mask Display: e = 0.06;c1 = [120 150 230]/255;c2 = ([120 150 230]+0)/383;c3 = ([120 150 230]+128)/383;patch([0 1 1 0],[0 0 1 1],c1);patch([0 1 1 1-e 1-e 0+e],[0 0 1 1-e 0+e 0+e],c2);patch([0 0 1 1-e 0+e 0+e],[0 1 1 1-e 1-e 0+e],c3);plot([0 1 1 0 0],[0 0 1 1 0]);disp('Weights');
  "IW{1,1}(29,:)'" : Constant  Value=[0.347471483882451692704051993132452480494976043701171875;-0.264940948232183115518267868537805043160915374755859375;2.8846574866064287334666005335748195648193359375;-0.35633156116019648607107228599488735198974609375;2.621864179071949241262018404086120426654815673828125]
      mask Display: e = 0.06;c1 = [120 150 230]/255;c2 = ([120 150 230]+0)/383;c3 = ([120 150 230]+128)/383;patch([0 1 1 0],[0 0 1 1],c1);patch([0 1 1 1-e 1-e 0+e],[0 0 1 1-e 0+e 0+e],c2);patch([0 0 1 1-e 0+e 0+e],[0 1 1 1-e 1-e 0+e],c3);plot([0 1 1 0 0],[0 0 1 1 0]);disp('Weights');
  "IW{1,1}(3,:)'" : Constant  Value=[1.143245178590432065135473749251104891300201416015625;1.921948926138987712164407639647834002971649169921875;-0.20962361997719825001951221565832383930683135986328125;2.6512263873439838590684303198941051959991455078125;2.01372348680733725956315538496710360050201416015625]
      mask Display: e = 0.06;c1 = [120 150 230]/255;c2 = ([120 150 230]+0)/383;c3 = ([120 150 230]+128)/383;patch([0 1 1 0],[0 0 1 1],c1);patch([0 1 1 1-e 1-e 0+e],[0 0 1 1-e 0+e 0+e],c2);patch([0 0 1 1-e 0+e 0+e],[0 1 1 1-e 1-e 0+e],c3);plot([0 1 1 0 0],[0 0 1 1 0]);disp('Weights');
  "IW{1,1}(30,:)'" : Constant  Value=[-0.287548751671504565496917393829789943993091583251953125;-2.700177108126438074719999349326826632022857666015625;1.5292950420203321737488977305474691092967987060546875;2.516261985862973116212515378720127046108245849609375;0.048854445846105730433261982170733972452580928802490234375]
      mask Display: e = 0.06;c1 = [120 150 230]/255;c2 = ([120 150 230]+0)/383;c3 = ([120 150 230]+128)/383;patch([0 1 1 0],[0 0 1 1],c1);patch([0 1 1 1-e 1-e 0+e],[0 0 1 1-e 0+e 0+e],c2);patch([0 0 1 1-e 0+e 0+e],[0 1 1 1-e 1-e 0+e],c3);plot([0 1 1 0 0],[0 0 1 1 0]);disp('Weights');
  "IW{1,1}(31,:)'" : Constant  Value=[-2.087429628019742633426858446910046041011810302734375;-2.044750179646072307804161027888767421245574951171875;1.113968921119980581835307020810432732105255126953125;1.6479645074589897024708307071705348789691925048828125;1.9865223121615238621728849466308020055294036865234375]
      mask Display: e = 0.06;c1 = [120 150 230]/255;c2 = ([120 150 230]+0)/383;c3 = ([120 150 230]+128)/383;patch([0 1 1 0],[0 0 1 1],c1);patch([0 1 1 1-e 1-e 0+e],[0 0 1 1-e 0+e 0+e],c2);patch([0 0 1 1-e 0+e 0+e],[0 1 1 1-e 1-e 0+e],c3);plot([0 1 1 0 0],[0 0 1 1 0]);disp('Weights');
  "IW{1,1}(32,:)'" : Constant  Value=[1.87104893530308036275755512178875505924224853515625;-1.9248100090369337777929104049690067768096923828125;0.346430285030580320526638615774572826921939849853515625;-2.01880672589062015731542487628757953643798828125;-2.431013230352395027011880301870405673980712890625]
      mask Display: e = 0.06;c1 = [120 150 230]/255;c2 = ([120 150 230]+0)/383;c3 = ([120 150 230]+128)/383;patch([0 1 1 0],[0 0 1 1],c1);patch([0 1 1 1-e 1-e 0+e],[0 0 1 1-e 0+e 0+e],c2);patch([0 0 1 1-e 0+e 0+e],[0 1 1 1-e 1-e 0+e],c3);plot([0 1 1 0 0],[0 0 1 1 0]);disp('Weights');
  "IW{1,1}(33,:)'" : Constant  Value=[0.897946046609744197297686696401797235012054443359375;-1.94223853981922189859687932766973972320556640625;0.0831455488009013310435335597503581084311008453369140625;-2.532379524187783115252159404917620122432708740234375;2.38599368043407533690469790599308907985687255859375]
      mask Display: e = 0.06;c1 = [120 150 230]/255;c2 = ([120 150 230]+0)/383;c3 = ([120 150 230]+128)/383;patch([0 1 1 0],[0 0 1 1],c1);patch([0 1 1 1-e 1-e 0+e],[0 0 1 1-e 0+e 0+e],c2);patch([0 0 1 1-e 0+e 0+e],[0 1 1 1-e 1-e 0+e],c3);plot([0 1 1 0 0],[0 0 1 1 0]);disp('Weights');
  "IW{1,1}(34,:)'" : Constant  Value=[-1.261045474665016374871129301027394831180572509765625;-0.926911149572756887238256240379996597766876220703125;1.9888580911138868945187141434871591627597808837890625;-2.36642603941480178519896071520633995532989501953125;-2.242858070972798767428457722417078912258148193359375]
      mask Display: e = 0.06;c1 = [120 150 230]/255;c2 = ([120 150 230]+0)/383;c3 = ([120 150 230]+128)/383;patch([0 1 1 0],[0 0 1 1],c1);patch([0 1 1 1-e 1-e 0+e],[0 0 1 1-e 0+e 0+e],c2);patch([0 0 1 1-e 0+e 0+e],[0 1 1 1-e 1-e 0+e],c3);plot([0 1 1 0 0],[0 0 1 1 0]);disp('Weights');
  "IW{1,1}(35,:)'" : Constant  Value=[2.453730519096621431884841513237915933132171630859375;2.34075323763534814958120477967895567417144775390625;-0.583200479703705365608357169548980891704559326171875;-1.8782492764311040644997774506919085979461669921875;-0.98996616653103763905363621233846060931682586669921875]
      mask Display: e = 0.06;c1 = [120 150 230]/255;c2 = ([120 150 230]+0)/383;c3 = ([120 150 230]+128)/383;patch([0 1 1 0],[0 0 1 1],c1);patch([0 1 1 1-e 1-e 0+e],[0 0 1 1-e 0+e 0+e],c2);patch([0 0 1 1-e 0+e 0+e],[0 1 1 1-e 1-e 0+e],c3);plot([0 1 1 0 0],[0 0 1 1 0]);disp('Weights');
  "IW{1,1}(36,:)'" : Constant  Value=[-2.344252727500263144833070327877067029476165771484375;0.242244160086804549703032307661487720906734466552734375;-0.28741896144086853670529535520472563803195953369140625;-2.461441149199450340034900364116765558719635009765625;2.112154278809963425800333425286225974559783935546875]
      mask Display: e = 0.06;c1 = [120 150 230]/255;c2 = ([120 150 230]+0)/383;c3 = ([120 150 230]+128)/383;patch([0 1 1 0],[0 0 1 1],c1);patch([0 1 1 1-e 1-e 0+e],[0 0 1 1-e 0+e 0+e],c2);patch([0 0 1 1-e 0+e 0+e],[0 1 1 1-e 1-e 0+e],c3);plot([0 1 1 0 0],[0 0 1 1 0]);disp('Weights');
  "IW{1,1}(37,:)'" : Constant  Value=[-1.8024492138226964055292000921326689422130584716796875;-2.621139785688090029225350008346140384674072265625;-2.885456840977262960024063431774266064167022705078125;0.98742550298160225441534976198454387485980987548828125;0.6510811084181806762671840260736644268035888671875]
      mask Display: e = 0.06;c1 = [120 150 230]/255;c2 = ([120 150 230]+0)/383;c3 = ([120 150 230]+128)/383;patch([0 1 1 0],[0 0 1 1],c1);patch([0 1 1 1-e 1-e 0+e],[0 0 1 1-e 0+e 0+e],c2);patch([0 0 1 1-e 0+e 0+e],[0 1 1 1-e 1-e 0+e],c3);plot([0 1 1 0 0],[0 0 1 1 0]);disp('Weights');
  "IW{1,1}(38,:)'" : Constant  Value=[-0.53406344289244900291890871812938712537288665771484375;-0.372312662481416978277337648250977508723735809326171875;2.001733730203743011344386104610748589038848876953125;-3.347794958119841179922104856814257800579071044921875;-0.12442444430880071626344118840279406867921352386474609375]
      mask Display: e = 0.06;c1 = [120 150 230]/255;c2 = ([120 150 230]+0)/383;c3 = ([120 150 230]+128)/383;patch([0 1 1 0],[0 0 1 1],c1);patch([0 1 1 1-e 1-e 0+e],[0 0 1 1-e 0+e 0+e],c2);patch([0 0 1 1-e 0+e 0+e],[0 1 1 1-e 1-e 0+e],c3);plot([0 1 1 0 0],[0 0 1 1 0]);disp('Weights');
  "IW{1,1}(39,:)'" : Constant  Value=[-2.685184995706407562465756200253963470458984375;1.9225202631329258995407371912733651697635650634765625;0.5845718754383286697162702694186009466648101806640625;-0.15437466017872936152599550041486509144306182861328125;-1.96828468175876292178827497991733253002166748046875]
      mask Display: e = 0.06;c1 = [120 150 230]/255;c2 = ([120 150 230]+0)/383;c3 = ([120 150 230]+128)/383;patch([0 1 1 0],[0 0 1 1],c1);patch([0 1 1 1-e 1-e 0+e],[0 0 1 1-e 0+e 0+e],c2);patch([0 0 1 1-e 0+e 0+e],[0 1 1 1-e 1-e 0+e],c3);plot([0 1 1 0 0],[0 0 1 1 0]);disp('Weights');
  "IW{1,1}(4,:)'" : Constant  Value=[-2.255988986497995174573816257179714739322662353515625;-1.3974011487435478162666413481929339468479156494140625;-0.377880608102285353577798332480597309768199920654296875;-0.2153211903565074025745929020558833144605159759521484375;-2.2005086413905718956129931029863655567169189453125]
      mask Display: e = 0.06;c1 = [120 150 230]/255;c2 = ([120 150 230]+0)/383;c3 = ([120 150 230]+128)/383;patch([0 1 1 0],[0 0 1 1],c1);patch([0 1 1 1-e 1-e 0+e],[0 0 1 1-e 0+e 0+e],c2);patch([0 0 1 1-e 0+e 0+e],[0 1 1 1-e 1-e 0+e],c3);plot([0 1 1 0 0],[0 0 1 1 0]);disp('Weights');
  "IW{1,1}(40,:)'" : Constant  Value=[-2.691738234710926658266316735534928739070892333984375;0.084302198784116100238605895356158725917339324951171875;-1.25604240663241117914594724425114691257476806640625;1.12866807561785176261537344544194638729095458984375;-3.097095389267380038944565967540256679058074951171875]
      mask Display: e = 0.06;c1 = [120 150 230]/255;c2 = ([120 150 230]+0)/383;c3 = ([120 150 230]+128)/383;patch([0 1 1 0],[0 0 1 1],c1);patch([0 1 1 1-e 1-e 0+e],[0 0 1 1-e 0+e 0+e],c2);patch([0 0 1 1-e 0+e 0+e],[0 1 1 1-e 1-e 0+e],c3);plot([0 1 1 0 0],[0 0 1 1 0]);disp('Weights');
  "IW{1,1}(41,:)'" : Constant  Value=[1.5800006966367423633101907398668117821216583251953125;0.80577388886448009230889510945416986942291259765625;1.4971894479810126110663759391172789037227630615234375;-3.012563096257026007407375800539739429950714111328125;-1.4539988475170704251837605625041760504245758056640625]
      mask Display: e = 0.06;c1 = [120 150 230]/255;c2 = ([120 150 230]+0)/383;c3 = ([120 150 230]+128)/383;patch([0 1 1 0],[0 0 1 1],c1);patch([0 1 1 1-e 1-e 0+e],[0 0 1 1-e 0+e 0+e],c2);patch([0 0 1 1-e 0+e 0+e],[0 1 1 1-e 1-e 0+e],c3);plot([0 1 1 0 0],[0 0 1 1 0]);disp('Weights');
  "IW{1,1}(42,:)'" : Constant  Value=[-2.078666283573972872744661799515597522258758544921875;1.8378462817637013504423748599947430193424224853515625;-2.146569149374906171345855909748934209346771240234375;-1.564781423302580076750700754928402602672576904296875;-1.9296249336185649081443216346087865531444549560546875]
      mask Display: e = 0.06;c1 = [120 150 230]/255;c2 = ([120 150 230]+0)/383;c3 = ([120 150 230]+128)/383;patch([0 1 1 0],[0 0 1 1],c1);patch([0 1 1 1-e 1-e 0+e],[0 0 1 1-e 0+e 0+e],c2);patch([0 0 1 1-e 0+e 0+e],[0 1 1 1-e 1-e 0+e],c3);plot([0 1 1 0 0],[0 0 1 1 0]);disp('Weights');
  "IW{1,1}(43,:)'" : Constant  Value=[-0.041868886409826049088689359223280916921794414520263671875;-1.100434294489212039280801036511547863483428955078125;-3.662290562486356204630055799498222768306732177734375;-1.6928272822481045256637344209593720734119415283203125;-1.5233696125344078353691656957380473613739013671875]
      mask Display: e = 0.06;c1 = [120 150 230]/255;c2 = ([120 150 230]+0)/383;c3 = ([120 150 230]+128)/383;patch([0 1 1 0],[0 0 1 1],c1);patch([0 1 1 1-e 1-e 0+e],[0 0 1 1-e 0+e 0+e],c2);patch([0 0 1 1-e 0+e 0+e],[0 1 1 1-e 1-e 0+e],c3);plot([0 1 1 0 0],[0 0 1 1 0]);disp('Weights');
  "IW{1,1}(44,:)'" : Constant  Value=[-1.351358981568508976778275609831325709819793701171875;1.7301309321201256974376292419037781655788421630859375;0.8655715247609740981005188587005250155925750732421875;-2.203729488097837307947202134528197348117828369140625;-2.67108654924279331766001632786355912685394287109375]
      mask Display: e = 0.06;c1 = [120 150 230]/255;c2 = ([120 150 230]+0)/383;c3 = ([120 150 230]+128)/383;patch([0 1 1 0],[0 0 1 1],c1);patch([0 1 1 1-e 1-e 0+e],[0 0 1 1-e 0+e 0+e],c2);patch([0 0 1 1-e 0+e 0+e],[0 1 1 1-e 1-e 0+e],c3);plot([0 1 1 0 0],[0 0 1 1 0]);disp('Weights');
  "IW{1,1}(45,:)'" : Constant  Value=[-0.27620272405489110223442139613325707614421844482421875;-2.571511704941709108851455312105827033519744873046875;1.207261930794726101368041781825013458728790283203125;-1.32817230169960165397924356511794030666351318359375;2.528946683674028417243562216754071414470672607421875]
      mask Display: e = 0.06;c1 = [120 150 230]/255;c2 = ([120 150 230]+0)/383;c3 = ([120 150 230]+128)/383;patch([0 1 1 0],[0 0 1 1],c1);patch([0 1 1 1-e 1-e 0+e],[0 0 1 1-e 0+e 0+e],c2);patch([0 0 1 1-e 0+e 0+e],[0 1 1 1-e 1-e 0+e],c3);plot([0 1 1 0 0],[0 0 1 1 0]);disp('Weights');
  "IW{1,1}(46,:)'" : Constant  Value=[1.991672404793582540349916598643176257610321044921875;-2.1614638988804042440960984094999730587005615234375;0.329429905379138132648364489796222187578678131103515625;1.42690731948713445120802134624682366847991943359375;2.235473113422168811581514091813005506992340087890625]
      mask Display: e = 0.06;c1 = [120 150 230]/255;c2 = ([120 150 230]+0)/383;c3 = ([120 150 230]+128)/383;patch([0 1 1 0],[0 0 1 1],c1);patch([0 1 1 1-e 1-e 0+e],[0 0 1 1-e 0+e 0+e],c2);patch([0 0 1 1-e 0+e 0+e],[0 1 1 1-e 1-e 0+e],c3);plot([0 1 1 0 0],[0 0 1 1 0]);disp('Weights');
  "IW{1,1}(47,:)'" : Constant  Value=[-2.046674605397942325879512281971983611583709716796875;-1.2894574149618860392507713186205364763736724853515625;2.49777489865225899023926103836856782436370849609375;-1.45027161159686546199054646422155201435089111328125;-1.951195306835929788036310128518380224704742431640625]
      mask Display: e = 0.06;c1 = [120 150 230]/255;c2 = ([120 150 230]+0)/383;c3 = ([120 150 230]+128)/383;patch([0 1 1 0],[0 0 1 1],c1);patch([0 1 1 1-e 1-e 0+e],[0 0 1 1-e 0+e 0+e],c2);patch([0 0 1 1-e 0+e 0+e],[0 1 1 1-e 1-e 0+e],c3);plot([0 1 1 0 0],[0 0 1 1 0]);disp('Weights');
  "IW{1,1}(48,:)'" : Constant  Value=[-3.215508015629357618792028006282635033130645751953125;1.882508977721418563788802202907390892505645751953125;0.8502225433282257771594458972685970366001129150390625;1.627103391776356655640256576589308679103851318359375;1.4876144376735374041942350231693126261234283447265625]
      mask Display: e = 0.06;c1 = [120 150 230]/255;c2 = ([120 150 230]+0)/383;c3 = ([120 150 230]+128)/383;patch([0 1 1 0],[0 0 1 1],c1);patch([0 1 1 1-e 1-e 0+e],[0 0 1 1-e 0+e 0+e],c2);patch([0 0 1 1-e 0+e 0+e],[0 1 1 1-e 1-e 0+e],c3);plot([0 1 1 0 0],[0 0 1 1 0]);disp('Weights');
  "IW{1,1}(49,:)'" : Constant  Value=[2.69473818726909808418668035301379859447479248046875;-0.6854109398767083138892530769226141273975372314453125;0.26698358610396943912945744159515015780925750732421875;0.439335881536435934879847309275646694004535675048828125;-2.815004253817865009779097817954607307910919189453125]
      mask Display: e = 0.06;c1 = [120 150 230]/255;c2 = ([120 150 230]+0)/383;c3 = ([120 150 230]+128)/383;patch([0 1 1 0],[0 0 1 1],c1);patch([0 1 1 1-e 1-e 0+e],[0 0 1 1-e 0+e 0+e],c2);patch([0 0 1 1-e 0+e 0+e],[0 1 1 1-e 1-e 0+e],c3);plot([0 1 1 0 0],[0 0 1 1 0]);disp('Weights');
  "IW{1,1}(5,:)'" : Constant  Value=[0.3361199802144045900575974883395247161388397216796875;-0.8725600063388194715940926471375860273838043212890625;-1.947194846989092287259381919284351170063018798828125;2.12266184946111824416448143892921507358551025390625;-2.67273686169964808101440212340094149112701416015625]
      mask Display: e = 0.06;c1 = [120 150 230]/255;c2 = ([120 150 230]+0)/383;c3 = ([120 150 230]+128)/383;patch([0 1 1 0],[0 0 1 1],c1);patch([0 1 1 1-e 1-e 0+e],[0 0 1 1-e 0+e 0+e],c2);patch([0 0 1 1-e 0+e 0+e],[0 1 1 1-e 1-e 0+e],c3);plot([0 1 1 0 0],[0 0 1 1 0]);disp('Weights');
  "IW{1,1}(50,:)'" : Constant  Value=[1.4728707489830747956460754721774719655513763427734375;3.282545895639286559486436090082861483097076416015625;-1.8586011492798732991360566302319057285785675048828125;0.55074563056140579675457047414965927600860595703125;0.92212684965951208226897506392560899257659912109375]
      mask Display: e = 0.06;c1 = [120 150 230]/255;c2 = ([120 150 230]+0)/383;c3 = ([120 150 230]+128)/383;patch([0 1 1 0],[0 0 1 1],c1);patch([0 1 1 1-e 1-e 0+e],[0 0 1 1-e 0+e 0+e],c2);patch([0 0 1 1-e 0+e 0+e],[0 1 1 1-e 1-e 0+e],c3);plot([0 1 1 0 0],[0 0 1 1 0]);disp('Weights');
  "IW{1,1}(51,:)'" : Constant  Value=[0.07719357127969088405716746592588606290519237518310546875;0.74452536898879062565725917011150158941745758056640625;-3.372372601445606132841703583835624158382415771484375;1.6549227905414938266659419241477735340595245361328125;1.2104880413318148679735486439312808215618133544921875]
      mask Display: e = 0.06;c1 = [120 150 230]/255;c2 = ([120 150 230]+0)/383;c3 = ([120 150 230]+128)/383;patch([0 1 1 0],[0 0 1 1],c1);patch([0 1 1 1-e 1-e 0+e],[0 0 1 1-e 0+e 0+e],c2);patch([0 0 1 1-e 0+e 0+e],[0 1 1 1-e 1-e 0+e],c3);plot([0 1 1 0 0],[0 0 1 1 0]);disp('Weights');
  "IW{1,1}(52,:)'" : Constant  Value=[0.08684792815205015503732255410795914940536022186279296875;-1.1129930578066040691709304155665449798107147216796875;1.38840090996371490206229282193817198276519775390625;1.777101770122089252623709398903883993625640869140625;-3.2705179202316347897294690483249723911285400390625]
      mask Display: e = 0.06;c1 = [120 150 230]/255;c2 = ([120 150 230]+0)/383;c3 = ([120 150 230]+128)/383;patch([0 1 1 0],[0 0 1 1],c1);patch([0 1 1 1-e 1-e 0+e],[0 0 1 1-e 0+e 0+e],c2);patch([0 0 1 1-e 0+e 0+e],[0 1 1 1-e 1-e 0+e],c3);plot([0 1 1 0 0],[0 0 1 1 0]);disp('Weights');
  "IW{1,1}(53,:)'" : Constant  Value=[-1.660282256637286568690115018398500978946685791015625;1.946430158175042723911474240594543516635894775390625;-1.4237489684752870910955380168161354959011077880859375;1.8065436032538413346770767020643688738346099853515625;-2.076079376825202604806008821469731628894805908203125]
      mask Display: e = 0.06;c1 = [120 150 230]/255;c2 = ([120 150 230]+0)/383;c3 = ([120 150 230]+128)/383;patch([0 1 1 0],[0 0 1 1],c1);patch([0 1 1 1-e 1-e 0+e],[0 0 1 1-e 0+e 0+e],c2);patch([0 0 1 1-e 0+e 0+e],[0 1 1 1-e 1-e 0+e],c3);plot([0 1 1 0 0],[0 0 1 1 0]);disp('Weights');
  "IW{1,1}(54,:)'" : Constant  Value=[2.332544414268094445930046276771463453769683837890625;1.9966020622769657943962329227360896766185760498046875;-0.944333137516137011147066004923544824123382568359375;-1.6321587190479458495673270590486936271190643310546875;-1.6488301760944448215440161220612935721874237060546875]
      mask Display: e = 0.06;c1 = [120 150 230]/255;c2 = ([120 150 230]+0)/383;c3 = ([120 150 230]+128)/383;patch([0 1 1 0],[0 0 1 1],c1);patch([0 1 1 1-e 1-e 0+e],[0 0 1 1-e 0+e 0+e],c2);patch([0 0 1 1-e 0+e 0+e],[0 1 1 1-e 1-e 0+e],c3);plot([0 1 1 0 0],[0 0 1 1 0]);disp('Weights');
  "IW{1,1}(55,:)'" : Constant  Value=[-1.202796464795855779783551042783074080944061279296875;2.0353788084778603462154933367855846881866455078125;-1.5523001452630180718728070132783614099025726318359375;1.5228198939627601848911808701814152300357818603515625;2.510376418153435817970375865115784108638763427734375]
      mask Display: e = 0.06;c1 = [120 150 230]/255;c2 = ([120 150 230]+0)/383;c3 = ([120 150 230]+128)/383;patch([0 1 1 0],[0 0 1 1],c1);patch([0 1 1 1-e 1-e 0+e],[0 0 1 1-e 0+e 0+e],c2);patch([0 0 1 1-e 0+e 0+e],[0 1 1 1-e 1-e 0+e],c3);plot([0 1 1 0 0],[0 0 1 1 0]);disp('Weights');
  "IW{1,1}(56,:)'" : Constant  Value=[0.9545602771989816215381097208592109382152557373046875;-2.075386496313333939411904793814755976200103759765625;0.356153177634801476614256898756138980388641357421875;-2.653631016772097783729122966178692877292633056640625;-1.8972041495235349994885609703487716615200042724609375]
      mask Display: e = 0.06;c1 = [120 150 230]/255;c2 = ([120 150 230]+0)/383;c3 = ([120 150 230]+128)/383;patch([0 1 1 0],[0 0 1 1],c1);patch([0 1 1 1-e 1-e 0+e],[0 0 1 1-e 0+e 0+e],c2);patch([0 0 1 1-e 0+e 0+e],[0 1 1 1-e 1-e 0+e],c3);plot([0 1 1 0 0],[0 0 1 1 0]);disp('Weights');
  "IW{1,1}(57,:)'" : Constant  Value=[-1.018524936671502789664600641117431223392486572265625;-1.6023078078374786148430075627402402460575103759765625;0.302736073581937159548971294498187489807605743408203125;-3.5612710219196941352493013255298137664794921875;0.53484151090266685013574488039012067019939422607421875]
      mask Display: e = 0.06;c1 = [120 150 230]/255;c2 = ([120 150 230]+0)/383;c3 = ([120 150 230]+128)/383;patch([0 1 1 0],[0 0 1 1],c1);patch([0 1 1 1-e 1-e 0+e],[0 0 1 1-e 0+e 0+e],c2);patch([0 0 1 1-e 0+e 0+e],[0 1 1 1-e 1-e 0+e],c3);plot([0 1 1 0 0],[0 0 1 1 0]);disp('Weights');
  "IW{1,1}(58,:)'" : Constant  Value=[-2.59125371588445485571128301671706140041351318359375;1.6142778907998238668852764021721668541431427001953125;1.66746722666992308603539640898816287517547607421875;-1.8980463385382251306765510889817960560321807861328125;0.26623096777012122959860107584972865879535675048828125]
      mask Display: e = 0.06;c1 = [120 150 230]/255;c2 = ([120 150 230]+0)/383;c3 = ([120 150 230]+128)/383;patch([0 1 1 0],[0 0 1 1],c1);patch([0 1 1 1-e 1-e 0+e],[0 0 1 1-e 0+e 0+e],c2);patch([0 0 1 1-e 0+e 0+e],[0 1 1 1-e 1-e 0+e],c3);plot([0 1 1 0 0],[0 0 1 1 0]);disp('Weights');
  "IW{1,1}(59,:)'" : Constant  Value=[0.363342446631722604255543274121009744703769683837890625;1.7295636933482849695309369053575210273265838623046875;2.7146172310438547725652824738062918186187744140625;-2.466167087873591068358791744685731828212738037109375;0.372135675689231393281630744240828789770603179931640625]
      mask Display: e = 0.06;c1 = [120 150 230]/255;c2 = ([120 150 230]+0)/383;c3 = ([120 150 230]+128)/383;patch([0 1 1 0],[0 0 1 1],c1);patch([0 1 1 1-e 1-e 0+e],[0 0 1 1-e 0+e 0+e],c2);patch([0 0 1 1-e 0+e 0+e],[0 1 1 1-e 1-e 0+e],c3);plot([0 1 1 0 0],[0 0 1 1 0]);disp('Weights');
  "IW{1,1}(6,:)'" : Constant  Value=[1.862602412614089875120271244668401777744293212890625;0.74182262669788678888238564468338154256343841552734375;-1.797652268455939950086985845700837671756744384765625;2.105421081926412529838898990419693291187286376953125;-2.1518726750176870865516320918686687946319580078125]
      mask Display: e = 0.06;c1 = [120 150 230]/255;c2 = ([120 150 230]+0)/383;c3 = ([120 150 230]+128)/383;patch([0 1 1 0],[0 0 1 1],c1);patch([0 1 1 1-e 1-e 0+e],[0 0 1 1-e 0+e 0+e],c2);patch([0 0 1 1-e 0+e 0+e],[0 1 1 1-e 1-e 0+e],c3);plot([0 1 1 0 0],[0 0 1 1 0]);disp('Weights');
  "IW{1,1}(60,:)'" : Constant  Value=[0.186078412682342764217224839740083552896976470947265625;0.060226494603996365284626079983354429714381694793701171875;2.480643399423552608595855417661368846893310546875;-2.7923174180781415998353622853755950927734375;-1.1968981133366707325649258564226329326629638671875]
      mask Display: e = 0.06;c1 = [120 150 230]/255;c2 = ([120 150 230]+0)/383;c3 = ([120 150 230]+128)/383;patch([0 1 1 0],[0 0 1 1],c1);patch([0 1 1 1-e 1-e 0+e],[0 0 1 1-e 0+e 0+e],c2);patch([0 0 1 1-e 0+e 0+e],[0 1 1 1-e 1-e 0+e],c3);plot([0 1 1 0 0],[0 0 1 1 0]);disp('Weights');
  "IW{1,1}(61,:)'" : Constant  Value=[-1.382218787066983534117525778128765523433685302734375;2.26694265198042188558247289620339870452880859375;2.00164329994165068882239211234264075756072998046875;2.31193372431855692639146582223474979400634765625;-0.52418041753604771582075727565097622573375701904296875]
      mask Display: e = 0.06;c1 = [120 150 230]/255;c2 = ([120 150 230]+0)/383;c3 = ([120 150 230]+128)/383;patch([0 1 1 0],[0 0 1 1],c1);patch([0 1 1 1-e 1-e 0+e],[0 0 1 1-e 0+e 0+e],c2);patch([0 0 1 1-e 0+e 0+e],[0 1 1 1-e 1-e 0+e],c3);plot([0 1 1 0 0],[0 0 1 1 0]);disp('Weights');
  "IW{1,1}(62,:)'" : Constant  Value=[-3.579883210363620893446068293997086584568023681640625;-0.7668349102747897827470069387345574796199798583984375;-3.206858794993651340377027736394666135311126708984375;-2.63008943876476397605301826843060553073883056640625;-2.2034602091735333573296884424053132534027099609375]
      mask Display: e = 0.06;c1 = [120 150 230]/255;c2 = ([120 150 230]+0)/383;c3 = ([120 150 230]+128)/383;patch([0 1 1 0],[0 0 1 1],c1);patch([0 1 1 1-e 1-e 0+e],[0 0 1 1-e 0+e 0+e],c2);patch([0 0 1 1-e 0+e 0+e],[0 1 1 1-e 1-e 0+e],c3);plot([0 1 1 0 0],[0 0 1 1 0]);disp('Weights');
  "IW{1,1}(63,:)'" : Constant  Value=[1.152349911141191451946497181779704988002777099609375;1.6151819772780038331205787471844814717769622802734375;1.1431314523937563532030026181018911302089691162109375;1.46923394444492938504254198051057755947113037109375;1.499268695532598005826230291859246790409088134765625]
      mask Display: e = 0.06;c1 = [120 150 230]/255;c2 = ([120 150 230]+0)/383;c3 = ([120 150 230]+128)/383;patch([0 1 1 0],[0 0 1 1],c1);patch([0 1 1 1-e 1-e 0+e],[0 0 1 1-e 0+e 0+e],c2);patch([0 0 1 1-e 0+e 0+e],[0 1 1 1-e 1-e 0+e],c3);plot([0 1 1 0 0],[0 0 1 1 0]);disp('Weights');
  "IW{1,1}(64,:)'" : Constant  Value=[-2.178580146596095001854109796113334596157073974609375;-0.337846499625516660803015156488982029259204864501953125;-2.636007618567875798731847680755890905857086181640625;0.2765098567179784527780839198385365307331085205078125;-2.716521246252523891229202490649186074733734130859375]
      mask Display: e = 0.06;c1 = [120 150 230]/255;c2 = ([120 150 230]+0)/383;c3 = ([120 150 230]+128)/383;patch([0 1 1 0],[0 0 1 1],c1);patch([0 1 1 1-e 1-e 0+e],[0 0 1 1-e 0+e 0+e],c2);patch([0 0 1 1-e 0+e 0+e],[0 1 1 1-e 1-e 0+e],c3);plot([0 1 1 0 0],[0 0 1 1 0]);disp('Weights');
  "IW{1,1}(65,:)'" : Constant  Value=[-1.4538893023745893540166207458241842687129974365234375;-0.1477148675785383835634689830840216018259525299072265625;-2.042351232308078134991546903620474040508270263671875;2.951453739694861244657886345521546900272369384765625;-0.90438123597553909949198214235366322100162506103515625]
      mask Display: e = 0.06;c1 = [120 150 230]/255;c2 = ([120 150 230]+0)/383;c3 = ([120 150 230]+128)/383;patch([0 1 1 0],[0 0 1 1],c1);patch([0 1 1 1-e 1-e 0+e],[0 0 1 1-e 0+e 0+e],c2);patch([0 0 1 1-e 0+e 0+e],[0 1 1 1-e 1-e 0+e],c3);plot([0 1 1 0 0],[0 0 1 1 0]);disp('Weights');
  "IW{1,1}(66,:)'" : Constant  Value=[1.5163391855807051289417586303898133337497711181640625;1.2230530478345895684100241851410828530788421630859375;-3.290606830374085856050214715651236474514007568359375;-1.2902588316715448701899049410712905228137969970703125;1.3257144643658513860629000191693194210529327392578125]
      mask Display: e = 0.06;c1 = [120 150 230]/255;c2 = ([120 150 230]+0)/383;c3 = ([120 150 230]+128)/383;patch([0 1 1 0],[0 0 1 1],c1);patch([0 1 1 1-e 1-e 0+e],[0 0 1 1-e 0+e 0+e],c2);patch([0 0 1 1-e 0+e 0+e],[0 1 1 1-e 1-e 0+e],c3);plot([0 1 1 0 0],[0 0 1 1 0]);disp('Weights');
  "IW{1,1}(67,:)'" : Constant  Value=[3.0329840399347371970861786394380033016204833984375;-0.64974789881056249640778332832269370555877685546875;0.90999971941552659782104228725074790418148040771484375;-1.8593848042737077808084222851903177797794342041015625;0.582027740172036178734060740680433809757232666015625]
      mask Display: e = 0.06;c1 = [120 150 230]/255;c2 = ([120 150 230]+0)/383;c3 = ([120 150 230]+128)/383;patch([0 1 1 0],[0 0 1 1],c1);patch([0 1 1 1-e 1-e 0+e],[0 0 1 1-e 0+e 0+e],c2);patch([0 0 1 1-e 0+e 0+e],[0 1 1 1-e 1-e 0+e],c3);plot([0 1 1 0 0],[0 0 1 1 0]);disp('Weights');
  "IW{1,1}(68,:)'" : Constant  Value=[0.61436467786152937353705283385352231562137603759765625;-0.74587872285974776698225241489126347005367279052734375;3.360371838563766200280724660842679440975189208984375;-2.275365728035167567355756546021439135074615478515625;-1.2084050006263382659454919121344573795795440673828125]
      mask Display: e = 0.06;c1 = [120 150 230]/255;c2 = ([120 150 230]+0)/383;c3 = ([120 150 230]+128)/383;patch([0 1 1 0],[0 0 1 1],c1);patch([0 1 1 1-e 1-e 0+e],[0 0 1 1-e 0+e 0+e],c2);patch([0 0 1 1-e 0+e 0+e],[0 1 1 1-e 1-e 0+e],c3);plot([0 1 1 0 0],[0 0 1 1 0]);disp('Weights');
  "IW{1,1}(69,:)'" : Constant  Value=[2.125739297809424943608291869168169796466827392578125;-2.4711487875843420880528356065042316913604736328125;0.550387426305261495684817418805323541164398193359375;0.352481068463185831518558188690803945064544677734375;2.62548247974996940001801704056560993194580078125]
      mask Display: e = 0.06;c1 = [120 150 230]/255;c2 = ([120 150 230]+0)/383;c3 = ([120 150 230]+128)/383;patch([0 1 1 0],[0 0 1 1],c1);patch([0 1 1 1-e 1-e 0+e],[0 0 1 1-e 0+e 0+e],c2);patch([0 0 1 1-e 0+e 0+e],[0 1 1 1-e 1-e 0+e],c3);plot([0 1 1 0 0],[0 0 1 1 0]);disp('Weights');
  "IW{1,1}(7,:)'" : Constant  Value=[0.53027268574343511264856942943879403173923492431640625;3.100126624093748173294216030626557767391204833984375;-0.84769033316173236780599609119235537946224212646484375;1.6780370270158082579570191228413023054599761962890625;1.5530189946341785844907690261607058346271514892578125]
      mask Display: e = 0.06;c1 = [120 150 230]/255;c2 = ([120 150 230]+0)/383;c3 = ([120 150 230]+128)/383;patch([0 1 1 0],[0 0 1 1],c1);patch([0 1 1 1-e 1-e 0+e],[0 0 1 1-e 0+e 0+e],c2);patch([0 0 1 1-e 0+e 0+e],[0 1 1 1-e 1-e 0+e],c3);plot([0 1 1 0 0],[0 0 1 1 0]);disp('Weights');
  "IW{1,1}(70,:)'" : Constant  Value=[1.379109656641277492639119373052380979061126708984375;1.70060726776623116762721110717393457889556884765625;-1.9248372715737203098029795000911690294742584228515625;-1.3727639766208046268047837656922638416290283203125;-2.640743959016759845326305367052555084228515625]
      mask Display: e = 0.06;c1 = [120 150 230]/255;c2 = ([120 150 230]+0)/383;c3 = ([120 150 230]+128)/383;patch([0 1 1 0],[0 0 1 1],c1);patch([0 1 1 1-e 1-e 0+e],[0 0 1 1-e 0+e 0+e],c2);patch([0 0 1 1-e 0+e 0+e],[0 1 1 1-e 1-e 0+e],c3);plot([0 1 1 0 0],[0 0 1 1 0]);disp('Weights');
  "IW{1,1}(71,:)'" : Constant  Value=[1.861090654995696258566795222577638924121856689453125;0.96100530008943341186977704637683928012847900390625;-0.147674289824659965564279673344572074711322784423828125;-2.9721947937070911649470872362144291400909423828125;-1.967325403602596001206848086440004408359527587890625]
      mask Display: e = 0.06;c1 = [120 150 230]/255;c2 = ([120 150 230]+0)/383;c3 = ([120 150 230]+128)/383;patch([0 1 1 0],[0 0 1 1],c1);patch([0 1 1 1-e 1-e 0+e],[0 0 1 1-e 0+e 0+e],c2);patch([0 0 1 1-e 0+e 0+e],[0 1 1 1-e 1-e 0+e],c3);plot([0 1 1 0 0],[0 0 1 1 0]);disp('Weights');
  "IW{1,1}(72,:)'" : Constant  Value=[1.0766386747599880902015456740627996623516082763671875;0.994433451718362615423529859981499612331390380859375;0.56903007963022134152453190836240537464618682861328125;-2.90597343098472382649788414710201323032379150390625;2.39608469003610213832189401728101074695587158203125]
      mask Display: e = 0.06;c1 = [120 150 230]/255;c2 = ([120 150 230]+0)/383;c3 = ([120 150 230]+128)/383;patch([0 1 1 0],[0 0 1 1],c1);patch([0 1 1 1-e 1-e 0+e],[0 0 1 1-e 0+e 0+e],c2);patch([0 0 1 1-e 0+e 0+e],[0 1 1 1-e 1-e 0+e],c3);plot([0 1 1 0 0],[0 0 1 1 0]);disp('Weights');
  "IW{1,1}(73,:)'" : Constant  Value=[2.569295499314750319541644785203970968723297119140625;1.7392787728378065192913481951109133660793304443359375;-2.120040461080260119075546754174865782260894775390625;0.44672341675726856546901899491786025464534759521484375;0.90786136747379286848769197604269720613956451416015625]
      mask Display: e = 0.06;c1 = [120 150 230]/255;c2 = ([120 150 230]+0)/383;c3 = ([120 150 230]+128)/383;patch([0 1 1 0],[0 0 1 1],c1);patch([0 1 1 1-e 1-e 0+e],[0 0 1 1-e 0+e 0+e],c2);patch([0 0 1 1-e 0+e 0+e],[0 1 1 1-e 1-e 0+e],c3);plot([0 1 1 0 0],[0 0 1 1 0]);disp('Weights');
  "IW{1,1}(74,:)'" : Constant  Value=[0.2410843191672728813568227224095608107745647430419921875;-1.881099753089581216869419222348369657993316650390625;-1.2048769389730382695091748246341012418270111083984375;3.16594548894001182048896225751377642154693603515625;1.32015540860223357100267094210721552371978759765625]
      mask Display: e = 0.06;c1 = [120 150 230]/255;c2 = ([120 150 230]+0)/383;c3 = ([120 150 230]+128)/383;patch([0 1 1 0],[0 0 1 1],c1);patch([0 1 1 1-e 1-e 0+e],[0 0 1 1-e 0+e 0+e],c2);patch([0 0 1 1-e 0+e 0+e],[0 1 1 1-e 1-e 0+e],c3);plot([0 1 1 0 0],[0 0 1 1 0]);disp('Weights');
  "IW{1,1}(75,:)'" : Constant  Value=[-0.004533253178902283721252164383486160659231245517730712890625;2.957028103069229363342174110584892332553863525390625;2.63818798737708792856437867158092558383941650390625;3.582282327212689576612092423602007329463958740234375;1.2788562509583820681058341506286524236202239990234375]
      mask Display: e = 0.06;c1 = [120 150 230]/255;c2 = ([120 150 230]+0)/383;c3 = ([120 150 230]+128)/383;patch([0 1 1 0],[0 0 1 1],c1);patch([0 1 1 1-e 1-e 0+e],[0 0 1 1-e 0+e 0+e],c2);patch([0 0 1 1-e 0+e 0+e],[0 1 1 1-e 1-e 0+e],c3);plot([0 1 1 0 0],[0 0 1 1 0]);disp('Weights');
  "IW{1,1}(76,:)'" : Constant  Value=[0.68915689185799322569181413200567476451396942138671875;2.0859944640921153080626027076505124568939208984375;0.133187411585790282941843543085269629955291748046875;-2.800408732222635865838356039603240787982940673828125;-2.461955615881926906496346418862231075763702392578125]
      mask Display: e = 0.06;c1 = [120 150 230]/255;c2 = ([120 150 230]+0)/383;c3 = ([120 150 230]+128)/383;patch([0 1 1 0],[0 0 1 1],c1);patch([0 1 1 1-e 1-e 0+e],[0 0 1 1-e 0+e 0+e],c2);patch([0 0 1 1-e 0+e 0+e],[0 1 1 1-e 1-e 0+e],c3);plot([0 1 1 0 0],[0 0 1 1 0]);disp('Weights');
  "IW{1,1}(77,:)'" : Constant  Value=[-0.51331085449792934749524420112720690667629241943359375;-1.4139951147156673005866878156666643917560577392578125;-2.08571060780179973193071418791078031063079833984375;0.95213002055752327112969624067773111164569854736328125;3.340767918342682829546674838638864457607269287109375]
      mask Display: e = 0.06;c1 = [120 150 230]/255;c2 = ([120 150 230]+0)/383;c3 = ([120 150 230]+128)/383;patch([0 1 1 0],[0 0 1 1],c1);patch([0 1 1 1-e 1-e 0+e],[0 0 1 1-e 0+e 0+e],c2);patch([0 0 1 1-e 0+e 0+e],[0 1 1 1-e 1-e 0+e],c3);plot([0 1 1 0 0],[0 0 1 1 0]);disp('Weights');
  "IW{1,1}(78,:)'" : Constant  Value=[-2.636413793821598350319845849298872053623199462890625;1.3371023018808632087939258781261742115020751953125;-1.254670938314593087170578655786812305450439453125;-1.13509823788870622962576817371882498264312744140625;2.14642147479142497701332104043103754520416259765625]
      mask Display: e = 0.06;c1 = [120 150 230]/255;c2 = ([120 150 230]+0)/383;c3 = ([120 150 230]+128)/383;patch([0 1 1 0],[0 0 1 1],c1);patch([0 1 1 1-e 1-e 0+e],[0 0 1 1-e 0+e 0+e],c2);patch([0 0 1 1-e 0+e 0+e],[0 1 1 1-e 1-e 0+e],c3);plot([0 1 1 0 0],[0 0 1 1 0]);disp('Weights');
  "IW{1,1}(79,:)'" : Constant  Value=[-1.4328055606349316963843421035562641918659210205078125;-4.16383415549495961016646106145344674587249755859375;-1.475061803045470743001033042673952877521514892578125;-4.183520482934678597075617290101945400238037109375;-1.54461703313509257640134819666855037212371826171875]
      mask Display: e = 0.06;c1 = [120 150 230]/255;c2 = ([120 150 230]+0)/383;c3 = ([120 150 230]+128)/383;patch([0 1 1 0],[0 0 1 1],c1);patch([0 1 1 1-e 1-e 0+e],[0 0 1 1-e 0+e 0+e],c2);patch([0 0 1 1-e 0+e 0+e],[0 1 1 1-e 1-e 0+e],c3);plot([0 1 1 0 0],[0 0 1 1 0]);disp('Weights');
  "IW{1,1}(8,:)'" : Constant  Value=[1.64687170454068887437415469321422278881072998046875;1.7328609038721245472203236204222775995731353759765625;0.03920347679454001810217533829927560873329639434814453125;-0.836110619735068727464977200725115835666656494140625;-3.149691522597845239062053224188275635242462158203125]
      mask Display: e = 0.06;c1 = [120 150 230]/255;c2 = ([120 150 230]+0)/383;c3 = ([120 150 230]+128)/383;patch([0 1 1 0],[0 0 1 1],c1);patch([0 1 1 1-e 1-e 0+e],[0 0 1 1-e 0+e 0+e],c2);patch([0 0 1 1-e 0+e 0+e],[0 1 1 1-e 1-e 0+e],c3);plot([0 1 1 0 0],[0 0 1 1 0]);disp('Weights');
  "IW{1,1}(80,:)'" : Constant  Value=[0.460337426016546535922913108151988126337528228759765625;-2.595453001849441054815770257846452295780181884765625;0.59574497361587186450293529560440219938755035400390625;0.5517470639745856164637416441109962761402130126953125;3.1571115140433345658266262034885585308074951171875]
      mask Display: e = 0.06;c1 = [120 150 230]/255;c2 = ([120 150 230]+0)/383;c3 = ([120 150 230]+128)/383;patch([0 1 1 0],[0 0 1 1],c1);patch([0 1 1 1-e 1-e 0+e],[0 0 1 1-e 0+e 0+e],c2);patch([0 0 1 1-e 0+e 0+e],[0 1 1 1-e 1-e 0+e],c3);plot([0 1 1 0 0],[0 0 1 1 0]);disp('Weights');
  "IW{1,1}(81,:)'" : Constant  Value=[-1.7623757377703810345082047206233255565166473388671875;-2.377714562075265547491653705947101116180419921875;-3.50309220634644447045502602122724056243896484375;-1.336425701124329901148257704335264861583709716796875;-1.4491037268014970162965937561239115893840789794921875]
      mask Display: e = 0.06;c1 = [120 150 230]/255;c2 = ([120 150 230]+0)/383;c3 = ([120 150 230]+128)/383;patch([0 1 1 0],[0 0 1 1],c1);patch([0 1 1 1-e 1-e 0+e],[0 0 1 1-e 0+e 0+e],c2);patch([0 0 1 1-e 0+e 0+e],[0 1 1 1-e 1-e 0+e],c3);plot([0 1 1 0 0],[0 0 1 1 0]);disp('Weights');
  "IW{1,1}(82,:)'" : Constant  Value=[-1.7195124807855701742909104723366908729076385498046875;2.57659001631784523311807788559235632419586181640625;1.229184306393993342254589151707477867603302001953125;0.17251889742772752445176820401684381067752838134765625;-2.275536910394797995849103244836442172527313232421875]
      mask Display: e = 0.06;c1 = [120 150 230]/255;c2 = ([120 150 230]+0)/383;c3 = ([120 150 230]+128)/383;patch([0 1 1 0],[0 0 1 1],c1);patch([0 1 1 1-e 1-e 0+e],[0 0 1 1-e 0+e 0+e],c2);patch([0 0 1 1-e 0+e 0+e],[0 1 1 1-e 1-e 0+e],c3);plot([0 1 1 0 0],[0 0 1 1 0]);disp('Weights');
  "IW{1,1}(83,:)'" : Constant  Value=[1.13100188152251224238398208399303257465362548828125;0.1515718224499743860267386708073900081217288970947265625;2.342396600720980881504829085315577685832977294921875;2.025719882687994743974968514521606266498565673828125;1.3934821217260964232309561339206993579864501953125]
      mask Display: e = 0.06;c1 = [120 150 230]/255;c2 = ([120 150 230]+0)/383;c3 = ([120 150 230]+128)/383;patch([0 1 1 0],[0 0 1 1],c1);patch([0 1 1 1-e 1-e 0+e],[0 0 1 1-e 0+e 0+e],c2);patch([0 0 1 1-e 0+e 0+e],[0 1 1 1-e 1-e 0+e],c3);plot([0 1 1 0 0],[0 0 1 1 0]);disp('Weights');
  "IW{1,1}(84,:)'" : Constant  Value=[-0.1398021365369450930149497480670106597244739532470703125;1.6314288886181060878044490891625173389911651611328125;-2.472339419866298015904249041341245174407958984375;-2.331286811072203146721903976867906749248504638671875;-2.058212253113019141181894156034104526042938232421875]
      mask Display: e = 0.06;c1 = [120 150 230]/255;c2 = ([120 150 230]+0)/383;c3 = ([120 150 230]+128)/383;patch([0 1 1 0],[0 0 1 1],c1);patch([0 1 1 1-e 1-e 0+e],[0 0 1 1-e 0+e 0+e],c2);patch([0 0 1 1-e 0+e 0+e],[0 1 1 1-e 1-e 0+e],c3);plot([0 1 1 0 0],[0 0 1 1 0]);disp('Weights');
  "IW{1,1}(85,:)'" : Constant  Value=[-0.1954260801736122099558912168504321016371250152587890625;-1.70051409594346925047148033627308905124664306640625;1.5189908199485844253473487697192467749118804931640625;-0.606933099530395647747127441107295453548431396484375;3.255853601882081616025743642239831387996673583984375]
      mask Display: e = 0.06;c1 = [120 150 230]/255;c2 = ([120 150 230]+0)/383;c3 = ([120 150 230]+128)/383;patch([0 1 1 0],[0 0 1 1],c1);patch([0 1 1 1-e 1-e 0+e],[0 0 1 1-e 0+e 0+e],c2);patch([0 0 1 1-e 0+e 0+e],[0 1 1 1-e 1-e 0+e],c3);plot([0 1 1 0 0],[0 0 1 1 0]);disp('Weights');
  "IW{1,1}(86,:)'" : Constant  Value=[-2.02978104718749552404233327251859009265899658203125;-1.4545616401343350876373961000354029238224029541015625;1.6077631804408536453365741181187331676483154296875;-2.117571420965165263083918034681119024753570556640625;-2.208968593494763155149485100992023944854736328125]
      mask Display: e = 0.06;c1 = [120 150 230]/255;c2 = ([120 150 230]+0)/383;c3 = ([120 150 230]+128)/383;patch([0 1 1 0],[0 0 1 1],c1);patch([0 1 1 1-e 1-e 0+e],[0 0 1 1-e 0+e 0+e],c2);patch([0 0 1 1-e 0+e 0+e],[0 1 1 1-e 1-e 0+e],c3);plot([0 1 1 0 0],[0 0 1 1 0]);disp('Weights');
  "IW{1,1}(87,:)'" : Constant  Value=[-2.781579261598347674322440070682205259799957275390625;-0.92119004869272946844915850306279025971889495849609375;1.18264532333702643285278099938295781612396240234375;-1.27322311256995135408942587673664093017578125;-2.212673756148517245634366190643049776554107666015625]
      mask Display: e = 0.06;c1 = [120 150 230]/255;c2 = ([120 150 230]+0)/383;c3 = ([120 150 230]+128)/383;patch([0 1 1 0],[0 0 1 1],c1);patch([0 1 1 1-e 1-e 0+e],[0 0 1 1-e 0+e 0+e],c2);patch([0 0 1 1-e 0+e 0+e],[0 1 1 1-e 1-e 0+e],c3);plot([0 1 1 0 0],[0 0 1 1 0]);disp('Weights');
  "IW{1,1}(88,:)'" : Constant  Value=[-0.274541074286096586920535855824709869921207427978515625;-0.125962662287786131276590140259941108524799346923828125;1.554518722554713239247803358011879026889801025390625;1.5817687613419340042497651666053570806980133056640625;-3.3677805367011028891965906950645148754119873046875]
      mask Display: e = 0.06;c1 = [120 150 230]/255;c2 = ([120 150 230]+0)/383;c3 = ([120 150 230]+128)/383;patch([0 1 1 0],[0 0 1 1],c1);patch([0 1 1 1-e 1-e 0+e],[0 0 1 1-e 0+e 0+e],c2);patch([0 0 1 1-e 0+e 0+e],[0 1 1 1-e 1-e 0+e],c3);plot([0 1 1 0 0],[0 0 1 1 0]);disp('Weights');
  "IW{1,1}(89,:)'" : Constant  Value=[1.1184216250138672155145513897878117859363555908203125;2.420265819725980094290207489393651485443115234375;-1.640291818206524254719624877907335758209228515625;-3.425260810589233262390962408971972763538360595703125;-0.019392746924284214038447515804364229552447795867919921875]
      mask Display: e = 0.06;c1 = [120 150 230]/255;c2 = ([120 150 230]+0)/383;c3 = ([120 150 230]+128)/383;patch([0 1 1 0],[0 0 1 1],c1);patch([0 1 1 1-e 1-e 0+e],[0 0 1 1-e 0+e 0+e],c2);patch([0 0 1 1-e 0+e 0+e],[0 1 1 1-e 1-e 0+e],c3);plot([0 1 1 0 0],[0 0 1 1 0]);disp('Weights');
  "IW{1,1}(9,:)'" : Constant  Value=[3.212705931361632405440786897088401019573211669921875;-0.96020023053292524739532609601155854761600494384765625;-1.3588661768745236013700150579097680747509002685546875;-0.70302818679995338069232957423082552850246429443359375;-1.6531174836374959991047717267065308988094329833984375]
      mask Display: e = 0.06;c1 = [120 150 230]/255;c2 = ([120 150 230]+0)/383;c3 = ([120 150 230]+128)/383;patch([0 1 1 0],[0 0 1 1],c1);patch([0 1 1 1-e 1-e 0+e],[0 0 1 1-e 0+e 0+e],c2);patch([0 0 1 1-e 0+e 0+e],[0 1 1 1-e 1-e 0+e],c3);plot([0 1 1 0 0],[0 0 1 1 0]);disp('Weights');
  "IW{1,1}(90,:)'" : Constant  Value=[1.8356326971010743509538087891996838152408599853515625;-2.670593193287970290583643873105756938457489013671875;-0.062382540155036060591786650775247835554182529449462890625;1.2907196628375821045864313418860547244548797607421875;2.42121385605272365637574694119393825531005859375]
      mask Display: e = 0.06;c1 = [120 150 230]/255;c2 = ([120 150 230]+0)/383;c3 = ([120 150 230]+128)/383;patch([0 1 1 0],[0 0 1 1],c1);patch([0 1 1 1-e 1-e 0+e],[0 0 1 1-e 0+e 0+e],c2);patch([0 0 1 1-e 0+e 0+e],[0 1 1 1-e 1-e 0+e],c3);plot([0 1 1 0 0],[0 0 1 1 0]);disp('Weights');
  "IW{1,1}(91,:)'" : Constant  Value=[2.556655006367939630962382580037228763103485107421875;-1.6890351304161990153573924544616602361202239990234375;-1.996380868338110570192611703532747924327850341796875;-1.09077902761064482461961233639158308506011962890625;1.7835738769437023965025446159415878355503082275390625]
      mask Display: e = 0.06;c1 = [120 150 230]/255;c2 = ([120 150 230]+0)/383;c3 = ([120 150 230]+128)/383;patch([0 1 1 0],[0 0 1 1],c1);patch([0 1 1 1-e 1-e 0+e],[0 0 1 1-e 0+e 0+e],c2);patch([0 0 1 1-e 0+e 0+e],[0 1 1 1-e 1-e 0+e],c3);plot([0 1 1 0 0],[0 0 1 1 0]);disp('Weights');
  "IW{1,1}(92,:)'" : Constant  Value=[4.8045726100939365466047092922963201999664306640625;2.243993851591511212717477974365465342998504638671875;0.289781467360619215956063499106676317751407623291015625;1.5762074004476236410710043855942785739898681640625;0.875735620636903799862693631439469754695892333984375]
      mask Display: e = 0.06;c1 = [120 150 230]/255;c2 = ([120 150 230]+0)/383;c3 = ([120 150 230]+128)/383;patch([0 1 1 0],[0 0 1 1],c1);patch([0 1 1 1-e 1-e 0+e],[0 0 1 1-e 0+e 0+e],c2);patch([0 0 1 1-e 0+e 0+e],[0 1 1 1-e 1-e 0+e],c3);plot([0 1 1 0 0],[0 0 1 1 0]);disp('Weights');
  "IW{1,1}(93,:)'" : Constant  Value=[-1.9273453321051714492995188265922479331493377685546875;-1.9666920811054711126786287422874011099338531494140625;-0.59777421208302372601650631622760556638240814208984375;-1.8429980952017703810241755491006188094615936279296875;1.6110355996164595904218685973319225013256072998046875]
      mask Display: e = 0.06;c1 = [120 150 230]/255;c2 = ([120 150 230]+0)/383;c3 = ([120 150 230]+128)/383;patch([0 1 1 0],[0 0 1 1],c1);patch([0 1 1 1-e 1-e 0+e],[0 0 1 1-e 0+e 0+e],c2);patch([0 0 1 1-e 0+e 0+e],[0 1 1 1-e 1-e 0+e],c3);plot([0 1 1 0 0],[0 0 1 1 0]);disp('Weights');
  "IW{1,1}(94,:)'" : Constant  Value=[3.01161981217870788896107114851474761962890625;-2.11259715034784445464310920215211808681488037109375;-1.5346701759988532476342015797854401171207427978515625;-0.427841549994739001050447768648155033588409423828125;0.74110699504773747126051830491633154451847076416015625]
      mask Display: e = 0.06;c1 = [120 150 230]/255;c2 = ([120 150 230]+0)/383;c3 = ([120 150 230]+128)/383;patch([0 1 1 0],[0 0 1 1],c1);patch([0 1 1 1-e 1-e 0+e],[0 0 1 1-e 0+e 0+e],c2);patch([0 0 1 1-e 0+e 0+e],[0 1 1 1-e 1-e 0+e],c3);plot([0 1 1 0 0],[0 0 1 1 0]);disp('Weights');
  "IW{1,1}(95,:)'" : Constant  Value=[-2.113830511609823492591431204346008598804473876953125;1.0611194917450699204408692821743898093700408935546875;1.70543971118566428657459255191497504711151123046875;-2.974320607310015684987547501805238425731658935546875;1.41022449815768613490263305720873177051544189453125]
      mask Display: e = 0.06;c1 = [120 150 230]/255;c2 = ([120 150 230]+0)/383;c3 = ([120 150 230]+128)/383;patch([0 1 1 0],[0 0 1 1],c1);patch([0 1 1 1-e 1-e 0+e],[0 0 1 1-e 0+e 0+e],c2);patch([0 0 1 1-e 0+e 0+e],[0 1 1 1-e 1-e 0+e],c3);plot([0 1 1 0 0],[0 0 1 1 0]);disp('Weights');
  "IW{1,1}(96,:)'" : Constant  Value=[2.4190494903748547272925861761905252933502197265625;-0.1173372096752915705319963990405085496604442596435546875;-0.53639218092687890315772847316111437976360321044921875;-1.67478950573099805154697605757974088191986083984375;-2.56475736354577943387766936211846768856048583984375]
      mask Display: e = 0.06;c1 = [120 150 230]/255;c2 = ([120 150 230]+0)/383;c3 = ([120 150 230]+128)/383;patch([0 1 1 0],[0 0 1 1],c1);patch([0 1 1 1-e 1-e 0+e],[0 0 1 1-e 0+e 0+e],c2);patch([0 0 1 1-e 0+e 0+e],[0 1 1 1-e 1-e 0+e],c3);plot([0 1 1 0 0],[0 0 1 1 0]);disp('Weights');
  "IW{1,1}(97,:)'" : Constant  Value=[1.090062281342060845901187349227257072925567626953125;0.417764995841854724911712537505081854760646820068359375;3.08237487433542955983512001694180071353912353515625;-2.21834273827344219398582936264574527740478515625;-0.11944239522601114711353176289776456542313098907470703125]
      mask Display: e = 0.06;c1 = [120 150 230]/255;c2 = ([120 150 230]+0)/383;c3 = ([120 150 230]+128)/383;patch([0 1 1 0],[0 0 1 1],c1);patch([0 1 1 1-e 1-e 0+e],[0 0 1 1-e 0+e 0+e],c2);patch([0 0 1 1-e 0+e 0+e],[0 1 1 1-e 1-e 0+e],c3);plot([0 1 1 0 0],[0 0 1 1 0]);disp('Weights');
  "IW{1,1}(98,:)'" : Constant  Value=[-1.5494576997131488393932841063360683619976043701171875;2.565440143228693070653889662935398519039154052734375;2.37847456795394140982580211129970848560333251953125;0.2315562742029566578594312886707484722137451171875;-1.7227308307915014662370367659605108201503753662109375]
      mask Display: e = 0.06;c1 = [120 150 230]/255;c2 = ([120 150 230]+0)/383;c3 = ([120 150 230]+128)/383;patch([0 1 1 0],[0 0 1 1],c1);patch([0 1 1 1-e 1-e 0+e],[0 0 1 1-e 0+e 0+e],c2);patch([0 0 1 1-e 0+e 0+e],[0 1 1 1-e 1-e 0+e],c3);plot([0 1 1 0 0],[0 0 1 1 0]);disp('Weights');
  "IW{1,1}(99,:)'" : Constant  Value=[-2.813672296872457678773571387864649295806884765625;1.7698191635106381713882228723377920687198638916015625;-1.32022442231484671282260023872368037700653076171875;-1.7947990437550334075211821982520632445812225341796875;-1.2283495741595498174092426779679954051971435546875]
      mask Display: e = 0.06;c1 = [120 150 230]/255;c2 = ([120 150 230]+0)/383;c3 = ([120 150 230]+128)/383;patch([0 1 1 0],[0 0 1 1],c1);patch([0 1 1 1-e 1-e 0+e],[0 0 1 1-e 0+e 0+e],c2);patch([0 0 1 1-e 0+e 0+e],[0 1 1 1-e 1-e 0+e],c3);plot([0 1 1 0 0],[0 0 1 1 0]);disp('Weights');
  Mux : Mux  Inputs=200
      mask Display: e = 0.06;c1 = [120 150 230]/255;c2 = ([120 150 230]+0)/383;c3 = ([120 150 230]+128)/383;patch([0 1 1 0],[0 0 1 1],c1);patch([0 1 1 1-e 1-e 0+e],[0 0 1 1-e 0+e 0+e],c2);patch([0 0 1 1-e 0+e 0+e],[0 1 1 1-e 1-e 0+e],c3);plot([0 1 1 0 0],[0 0 1 1 0]);disp('Mux');
  dotprod{1..200} (200 alike) : neural/Weight Functions/dotprod
  "iz{1,1}" : Outport
      mask Display: e = 0.06;c1 = [120 230 180]/255;c2 = ([120 230 180]+0)/(256+128);c3 = ([120 230 180]+128)/(256+128);patch([0 1 1 0],[0 0 1 1],c1);patch([0 1 1 1-e 1-e 0+e],[0 0 1 1-e 0+e 0+e],c2);patch([0 0 1 1-e 0+e 0+e],[0 1 1 1-e 1-e 0+e],c3);plot([0 1 1 0 0],[0 0 1 1 0]);
  wires:
  "IW{1,1}(1,:)'"/1 -> dotprod1/1
  "pd{1,1}"/1 -> dotprod1/2, dotprod2/2, dotprod3/2, dotprod4/2, dotprod5/2, dotprod6/2, dotprod7/2, dotprod8/2, dotprod9/2, dotprod10/2, dotprod11/2, dotprod12/2, dotprod13/2, dotprod14/2, dotprod15/2, dotprod16/2, dotprod17/2, dotprod18/2, dotprod19/2, dotprod20/2, dotprod21/2, dotprod22/2, dotprod23/2, dotprod24/2, dotprod25/2, dotprod26/2, dotprod27/2, dotprod28/2, dotprod29/2, dotprod30/2, dotprod31/2, dotprod32/2, dotprod33/2, dotprod34/2, dotprod35/2, dotprod36/2, dotprod37/2, dotprod38/2, dotprod39/2, dotprod40/2, dotprod41/2, dotprod42/2, dotprod43/2, dotprod44/2, dotprod45/2, dotprod46/2, dotprod47/2, dotprod48/2, dotprod49/2, dotprod50/2, dotprod51/2, dotprod52/2, dotprod53/2, dotprod54/2, dotprod55/2, dotprod56/2, dotprod57/2, dotprod58/2, dotprod59/2, dotprod60/2, dotprod61/2, dotprod62/2, dotprod63/2, dotprod64/2, dotprod65/2, dotprod66/2, dotprod67/2, dotprod68/2, dotprod69/2, dotprod70/2, dotprod71/2, dotprod72/2, dotprod73/2, dotprod74/2, dotprod75/2, dotprod76/2, dotprod77/2, dotprod78/2, dotprod79/2, dotprod80/2, dotprod81/2, dotprod82/2, dotprod83/2, dotprod84/2, dotprod85/2, dotprod86/2, dotprod87/2, dotprod88/2, dotprod89/2, dotprod90/2, dotprod91/2, dotprod92/2, dotprod93/2, dotprod94/2, dotprod95/2, dotprod96/2, dotprod97/2, dotprod98/2, dotprod99/2, dotprod100/2, dotprod101/2, dotprod102/2, dotprod103/2, dotprod104/2, dotprod105/2, dotprod106/2, dotprod107/2, dotprod108/2, dotprod109/2, dotprod110/2, dotprod111/2, dotprod112/2, dotprod113/2, dotprod114/2, dotprod115/2, dotprod116/2, dotprod117/2, dotprod118/2, dotprod119/2, dotprod120/2, dotprod121/2, dotprod122/2, dotprod123/2, dotprod124/2, dotprod125/2, dotprod126/2, dotprod127/2, dotprod128/2, dotprod129/2, dotprod130/2, dotprod131/2, dotprod132/2, dotprod133/2, dotprod134/2, dotprod135/2, dotprod136/2, dotprod137/2, dotprod138/2, dotprod139/2, dotprod140/2, dotprod141/2, dotprod142/2, dotprod143/2, dotprod144/2, dotprod145/2, dotprod146/2, dotprod147/2, dotprod148/2, dotprod149/2, dotprod150/2, dotprod151/2, dotprod152/2, dotprod153/2, dotprod154/2, dotprod155/2, dotprod156/2, dotprod157/2, dotprod158/2, dotprod159/2, dotprod160/2, dotprod161/2, dotprod162/2, dotprod163/2, dotprod164/2, dotprod165/2, dotprod166/2, dotprod167/2, dotprod168/2, dotprod169/2, dotprod170/2, dotprod171/2, dotprod172/2, dotprod173/2, dotprod174/2, dotprod175/2, dotprod176/2, dotprod177/2, dotprod178/2, dotprod179/2, dotprod180/2, dotprod181/2, dotprod182/2, dotprod183/2, dotprod184/2, dotprod185/2, dotprod186/2, dotprod187/2, dotprod188/2, dotprod189/2, dotprod190/2, dotprod191/2, dotprod192/2, dotprod193/2, dotprod194/2, dotprod195/2, dotprod196/2, dotprod197/2, dotprod198/2, dotprod199/2, dotprod200/2
  dotprod1/1 -> Mux/1
  "IW{1,1}(2,:)'"/1 -> dotprod2/1
  dotprod2/1 -> Mux/2
  "IW{1,1}(3,:)'"/1 -> dotprod3/1
  dotprod3/1 -> Mux/3
  "IW{1,1}(4,:)'"/1 -> dotprod4/1
  dotprod4/1 -> Mux/4
  "IW{1,1}(5,:)'"/1 -> dotprod5/1
  dotprod5/1 -> Mux/5
  "IW{1,1}(6,:)'"/1 -> dotprod6/1
  dotprod6/1 -> Mux/6
  "IW{1,1}(7,:)'"/1 -> dotprod7/1
  dotprod7/1 -> Mux/7
  "IW{1,1}(8,:)'"/1 -> dotprod8/1
  dotprod8/1 -> Mux/8
  "IW{1,1}(9,:)'"/1 -> dotprod9/1
  dotprod9/1 -> Mux/9
  "IW{1,1}(10,:)'"/1 -> dotprod10/1
  dotprod10/1 -> Mux/10
  "IW{1,1}(11,:)'"/1 -> dotprod11/1
  dotprod11/1 -> Mux/11
  "IW{1,1}(12,:)'"/1 -> dotprod12/1
  dotprod12/1 -> Mux/12
  "IW{1,1}(13,:)'"/1 -> dotprod13/1
  dotprod13/1 -> Mux/13
  "IW{1,1}(14,:)'"/1 -> dotprod14/1
  dotprod14/1 -> Mux/14
  "IW{1,1}(15,:)'"/1 -> dotprod15/1
  dotprod15/1 -> Mux/15
  "IW{1,1}(16,:)'"/1 -> dotprod16/1
  dotprod16/1 -> Mux/16
  "IW{1,1}(17,:)'"/1 -> dotprod17/1
  dotprod17/1 -> Mux/17
  "IW{1,1}(18,:)'"/1 -> dotprod18/1
  dotprod18/1 -> Mux/18
  "IW{1,1}(19,:)'"/1 -> dotprod19/1
  dotprod19/1 -> Mux/19
  "IW{1,1}(20,:)'"/1 -> dotprod20/1
  dotprod20/1 -> Mux/20
  "IW{1,1}(21,:)'"/1 -> dotprod21/1
  dotprod21/1 -> Mux/21
  "IW{1,1}(22,:)'"/1 -> dotprod22/1
  dotprod22/1 -> Mux/22
  "IW{1,1}(23,:)'"/1 -> dotprod23/1
  dotprod23/1 -> Mux/23
  "IW{1,1}(24,:)'"/1 -> dotprod24/1
  dotprod24/1 -> Mux/24
  "IW{1,1}(25,:)'"/1 -> dotprod25/1
  dotprod25/1 -> Mux/25
  "IW{1,1}(26,:)'"/1 -> dotprod26/1
  dotprod26/1 -> Mux/26
  "IW{1,1}(27,:)'"/1 -> dotprod27/1
  dotprod27/1 -> Mux/27
  "IW{1,1}(28,:)'"/1 -> dotprod28/1
  dotprod28/1 -> Mux/28
  "IW{1,1}(29,:)'"/1 -> dotprod29/1
  dotprod29/1 -> Mux/29
  "IW{1,1}(30,:)'"/1 -> dotprod30/1
  dotprod30/1 -> Mux/30
  "IW{1,1}(31,:)'"/1 -> dotprod31/1
  dotprod31/1 -> Mux/31
  "IW{1,1}(32,:)'"/1 -> dotprod32/1
  dotprod32/1 -> Mux/32
  "IW{1,1}(33,:)'"/1 -> dotprod33/1
  dotprod33/1 -> Mux/33
  "IW{1,1}(34,:)'"/1 -> dotprod34/1
  dotprod34/1 -> Mux/34
  "IW{1,1}(35,:)'"/1 -> dotprod35/1
  dotprod35/1 -> Mux/35
  "IW{1,1}(36,:)'"/1 -> dotprod36/1
  dotprod36/1 -> Mux/36
  "IW{1,1}(37,:)'"/1 -> dotprod37/1
  dotprod37/1 -> Mux/37
  "IW{1,1}(38,:)'"/1 -> dotprod38/1
  dotprod38/1 -> Mux/38
  "IW{1,1}(39,:)'"/1 -> dotprod39/1
  dotprod39/1 -> Mux/39
  "IW{1,1}(40,:)'"/1 -> dotprod40/1
  dotprod40/1 -> Mux/40
  "IW{1,1}(41,:)'"/1 -> dotprod41/1
  dotprod41/1 -> Mux/41
  "IW{1,1}(42,:)'"/1 -> dotprod42/1
  dotprod42/1 -> Mux/42
  "IW{1,1}(43,:)'"/1 -> dotprod43/1
  dotprod43/1 -> Mux/43
  "IW{1,1}(44,:)'"/1 -> dotprod44/1
  dotprod44/1 -> Mux/44
  "IW{1,1}(45,:)'"/1 -> dotprod45/1
  dotprod45/1 -> Mux/45
  "IW{1,1}(46,:)'"/1 -> dotprod46/1
  dotprod46/1 -> Mux/46
  "IW{1,1}(47,:)'"/1 -> dotprod47/1
  dotprod47/1 -> Mux/47
  "IW{1,1}(48,:)'"/1 -> dotprod48/1
  dotprod48/1 -> Mux/48
  "IW{1,1}(49,:)'"/1 -> dotprod49/1
  dotprod49/1 -> Mux/49
  "IW{1,1}(50,:)'"/1 -> dotprod50/1
  dotprod50/1 -> Mux/50
  "IW{1,1}(51,:)'"/1 -> dotprod51/1
  dotprod51/1 -> Mux/51
  "IW{1,1}(52,:)'"/1 -> dotprod52/1
  dotprod52/1 -> Mux/52
  "IW{1,1}(53,:)'"/1 -> dotprod53/1
  dotprod53/1 -> Mux/53
  "IW{1,1}(54,:)'"/1 -> dotprod54/1
  dotprod54/1 -> Mux/54
  "IW{1,1}(55,:)'"/1 -> dotprod55/1
  dotprod55/1 -> Mux/55
  "IW{1,1}(56,:)'"/1 -> dotprod56/1
  dotprod56/1 -> Mux/56
  "IW{1,1}(57,:)'"/1 -> dotprod57/1
  dotprod57/1 -> Mux/57
  "IW{1,1}(58,:)'"/1 -> dotprod58/1
  dotprod58/1 -> Mux/58
  "IW{1,1}(59,:)'"/1 -> dotprod59/1
  dotprod59/1 -> Mux/59
  "IW{1,1}(60,:)'"/1 -> dotprod60/1
  dotprod60/1 -> Mux/60
  "IW{1,1}(61,:)'"/1 -> dotprod61/1
  dotprod61/1 -> Mux/61
  "IW{1,1}(62,:)'"/1 -> dotprod62/1
  dotprod62/1 -> Mux/62
  "IW{1,1}(63,:)'"/1 -> dotprod63/1
  dotprod63/1 -> Mux/63
  "IW{1,1}(64,:)'"/1 -> dotprod64/1
  dotprod64/1 -> Mux/64
  "IW{1,1}(65,:)'"/1 -> dotprod65/1
  dotprod65/1 -> Mux/65
  "IW{1,1}(66,:)'"/1 -> dotprod66/1
  dotprod66/1 -> Mux/66
  "IW{1,1}(67,:)'"/1 -> dotprod67/1
  dotprod67/1 -> Mux/67
  "IW{1,1}(68,:)'"/1 -> dotprod68/1
  dotprod68/1 -> Mux/68
  "IW{1,1}(69,:)'"/1 -> dotprod69/1
  dotprod69/1 -> Mux/69
  "IW{1,1}(70,:)'"/1 -> dotprod70/1
  dotprod70/1 -> Mux/70
  "IW{1,1}(71,:)'"/1 -> dotprod71/1
  dotprod71/1 -> Mux/71
  "IW{1,1}(72,:)'"/1 -> dotprod72/1
  dotprod72/1 -> Mux/72
  "IW{1,1}(73,:)'"/1 -> dotprod73/1
  dotprod73/1 -> Mux/73
  "IW{1,1}(74,:)'"/1 -> dotprod74/1
  dotprod74/1 -> Mux/74
  "IW{1,1}(75,:)'"/1 -> dotprod75/1
  dotprod75/1 -> Mux/75
  "IW{1,1}(76,:)'"/1 -> dotprod76/1
  dotprod76/1 -> Mux/76
  "IW{1,1}(77,:)'"/1 -> dotprod77/1
  dotprod77/1 -> Mux/77
  "IW{1,1}(78,:)'"/1 -> dotprod78/1
  dotprod78/1 -> Mux/78
  "IW{1,1}(79,:)'"/1 -> dotprod79/1
  dotprod79/1 -> Mux/79
  "IW{1,1}(80,:)'"/1 -> dotprod80/1
  dotprod80/1 -> Mux/80
  "IW{1,1}(81,:)'"/1 -> dotprod81/1
  dotprod81/1 -> Mux/81
  "IW{1,1}(82,:)'"/1 -> dotprod82/1
  dotprod82/1 -> Mux/82
  "IW{1,1}(83,:)'"/1 -> dotprod83/1
  dotprod83/1 -> Mux/83
  "IW{1,1}(84,:)'"/1 -> dotprod84/1
  dotprod84/1 -> Mux/84
  "IW{1,1}(85,:)'"/1 -> dotprod85/1
  dotprod85/1 -> Mux/85
  "IW{1,1}(86,:)'"/1 -> dotprod86/1
  dotprod86/1 -> Mux/86
  "IW{1,1}(87,:)'"/1 -> dotprod87/1
  dotprod87/1 -> Mux/87
  "IW{1,1}(88,:)'"/1 -> dotprod88/1
  dotprod88/1 -> Mux/88
  "IW{1,1}(89,:)'"/1 -> dotprod89/1
  dotprod89/1 -> Mux/89
  "IW{1,1}(90,:)'"/1 -> dotprod90/1
  dotprod90/1 -> Mux/90
  "IW{1,1}(91,:)'"/1 -> dotprod91/1
  dotprod91/1 -> Mux/91
  "IW{1,1}(92,:)'"/1 -> dotprod92/1
  dotprod92/1 -> Mux/92
  "IW{1,1}(93,:)'"/1 -> dotprod93/1
  dotprod93/1 -> Mux/93
  "IW{1,1}(94,:)'"/1 -> dotprod94/1
  dotprod94/1 -> Mux/94
  "IW{1,1}(95,:)'"/1 -> dotprod95/1
  dotprod95/1 -> Mux/95
  "IW{1,1}(96,:)'"/1 -> dotprod96/1
  dotprod96/1 -> Mux/96
  "IW{1,1}(97,:)'"/1 -> dotprod97/1
  dotprod97/1 -> Mux/97
  "IW{1,1}(98,:)'"/1 -> dotprod98/1
  dotprod98/1 -> Mux/98
  "IW{1,1}(99,:)'"/1 -> dotprod99/1
  dotprod99/1 -> Mux/99
  "IW{1,1}(100,:)'"/1 -> dotprod100/1
  dotprod100/1 -> Mux/100
  "IW{1,1}(101,:)'"/1 -> dotprod101/1
  dotprod101/1 -> Mux/101
  "IW{1,1}(102,:)'"/1 -> dotprod102/1
  dotprod102/1 -> Mux/102
  "IW{1,1}(103,:)'"/1 -> dotprod103/1
  dotprod103/1 -> Mux/103
  "IW{1,1}(104,:)'"/1 -> dotprod104/1
  dotprod104/1 -> Mux/104
  "IW{1,1}(105,:)'"/1 -> dotprod105/1
  dotprod105/1 -> Mux/105
  "IW{1,1}(106,:)'"/1 -> dotprod106/1
  dotprod106/1 -> Mux/106
  "IW{1,1}(107,:)'"/1 -> dotprod107/1
  dotprod107/1 -> Mux/107
  "IW{1,1}(108,:)'"/1 -> dotprod108/1
  dotprod108/1 -> Mux/108
  "IW{1,1}(109,:)'"/1 -> dotprod109/1
  dotprod109/1 -> Mux/109
  "IW{1,1}(110,:)'"/1 -> dotprod110/1
  dotprod110/1 -> Mux/110
  "IW{1,1}(111,:)'"/1 -> dotprod111/1
  dotprod111/1 -> Mux/111
  "IW{1,1}(112,:)'"/1 -> dotprod112/1
  dotprod112/1 -> Mux/112
  "IW{1,1}(113,:)'"/1 -> dotprod113/1
  dotprod113/1 -> Mux/113
  "IW{1,1}(114,:)'"/1 -> dotprod114/1
  dotprod114/1 -> Mux/114
  "IW{1,1}(115,:)'"/1 -> dotprod115/1
  dotprod115/1 -> Mux/115
  "IW{1,1}(116,:)'"/1 -> dotprod116/1
  dotprod116/1 -> Mux/116
  "IW{1,1}(117,:)'"/1 -> dotprod117/1
  dotprod117/1 -> Mux/117
  "IW{1,1}(118,:)'"/1 -> dotprod118/1
  dotprod118/1 -> Mux/118
  "IW{1,1}(119,:)'"/1 -> dotprod119/1
  dotprod119/1 -> Mux/119
  "IW{1,1}(120,:)'"/1 -> dotprod120/1
  dotprod120/1 -> Mux/120
  "IW{1,1}(121,:)'"/1 -> dotprod121/1
  dotprod121/1 -> Mux/121
  "IW{1,1}(122,:)'"/1 -> dotprod122/1
  dotprod122/1 -> Mux/122
  "IW{1,1}(123,:)'"/1 -> dotprod123/1
  dotprod123/1 -> Mux/123
  "IW{1,1}(124,:)'"/1 -> dotprod124/1
  dotprod124/1 -> Mux/124
  "IW{1,1}(125,:)'"/1 -> dotprod125/1
  dotprod125/1 -> Mux/125
  "IW{1,1}(126,:)'"/1 -> dotprod126/1
  dotprod126/1 -> Mux/126
  "IW{1,1}(127,:)'"/1 -> dotprod127/1
  dotprod127/1 -> Mux/127
  "IW{1,1}(128,:)'"/1 -> dotprod128/1
  dotprod128/1 -> Mux/128
  "IW{1,1}(129,:)'"/1 -> dotprod129/1
  dotprod129/1 -> Mux/129
  "IW{1,1}(130,:)'"/1 -> dotprod130/1
  dotprod130/1 -> Mux/130
  "IW{1,1}(131,:)'"/1 -> dotprod131/1
  dotprod131/1 -> Mux/131
  "IW{1,1}(132,:)'"/1 -> dotprod132/1
  dotprod132/1 -> Mux/132
  "IW{1,1}(133,:)'"/1 -> dotprod133/1
  dotprod133/1 -> Mux/133
  "IW{1,1}(134,:)'"/1 -> dotprod134/1
  dotprod134/1 -> Mux/134
  "IW{1,1}(135,:)'"/1 -> dotprod135/1
  dotprod135/1 -> Mux/135
  "IW{1,1}(136,:)'"/1 -> dotprod136/1
  dotprod136/1 -> Mux/136
  "IW{1,1}(137,:)'"/1 -> dotprod137/1
  dotprod137/1 -> Mux/137
  "IW{1,1}(138,:)'"/1 -> dotprod138/1
  dotprod138/1 -> Mux/138
  "IW{1,1}(139,:)'"/1 -> dotprod139/1
  dotprod139/1 -> Mux/139
  "IW{1,1}(140,:)'"/1 -> dotprod140/1
  dotprod140/1 -> Mux/140
  "IW{1,1}(141,:)'"/1 -> dotprod141/1
  dotprod141/1 -> Mux/141
  "IW{1,1}(142,:)'"/1 -> dotprod142/1
  dotprod142/1 -> Mux/142
  "IW{1,1}(143,:)'"/1 -> dotprod143/1
  dotprod143/1 -> Mux/143
  "IW{1,1}(144,:)'"/1 -> dotprod144/1
  dotprod144/1 -> Mux/144
  "IW{1,1}(145,:)'"/1 -> dotprod145/1
  dotprod145/1 -> Mux/145
  "IW{1,1}(146,:)'"/1 -> dotprod146/1
  dotprod146/1 -> Mux/146
  "IW{1,1}(147,:)'"/1 -> dotprod147/1
  dotprod147/1 -> Mux/147
  "IW{1,1}(148,:)'"/1 -> dotprod148/1
  dotprod148/1 -> Mux/148
  "IW{1,1}(149,:)'"/1 -> dotprod149/1
  dotprod149/1 -> Mux/149
  "IW{1,1}(150,:)'"/1 -> dotprod150/1
  dotprod150/1 -> Mux/150
  "IW{1,1}(151,:)'"/1 -> dotprod151/1
  dotprod151/1 -> Mux/151
  "IW{1,1}(152,:)'"/1 -> dotprod152/1
  dotprod152/1 -> Mux/152
  "IW{1,1}(153,:)'"/1 -> dotprod153/1
  dotprod153/1 -> Mux/153
  "IW{1,1}(154,:)'"/1 -> dotprod154/1
  dotprod154/1 -> Mux/154
  "IW{1,1}(155,:)'"/1 -> dotprod155/1
  dotprod155/1 -> Mux/155
  "IW{1,1}(156,:)'"/1 -> dotprod156/1
  dotprod156/1 -> Mux/156
  "IW{1,1}(157,:)'"/1 -> dotprod157/1
  dotprod157/1 -> Mux/157
  "IW{1,1}(158,:)'"/1 -> dotprod158/1
  dotprod158/1 -> Mux/158
  "IW{1,1}(159,:)'"/1 -> dotprod159/1
  dotprod159/1 -> Mux/159
  "IW{1,1}(160,:)'"/1 -> dotprod160/1
  dotprod160/1 -> Mux/160
  "IW{1,1}(161,:)'"/1 -> dotprod161/1
  dotprod161/1 -> Mux/161
  "IW{1,1}(162,:)'"/1 -> dotprod162/1
  dotprod162/1 -> Mux/162
  "IW{1,1}(163,:)'"/1 -> dotprod163/1
  dotprod163/1 -> Mux/163
  "IW{1,1}(164,:)'"/1 -> dotprod164/1
  dotprod164/1 -> Mux/164
  "IW{1,1}(165,:)'"/1 -> dotprod165/1
  dotprod165/1 -> Mux/165
  "IW{1,1}(166,:)'"/1 -> dotprod166/1
  dotprod166/1 -> Mux/166
  "IW{1,1}(167,:)'"/1 -> dotprod167/1
  dotprod167/1 -> Mux/167
  "IW{1,1}(168,:)'"/1 -> dotprod168/1
  dotprod168/1 -> Mux/168
  "IW{1,1}(169,:)'"/1 -> dotprod169/1
  dotprod169/1 -> Mux/169
  "IW{1,1}(170,:)'"/1 -> dotprod170/1
  dotprod170/1 -> Mux/170
  "IW{1,1}(171,:)'"/1 -> dotprod171/1
  dotprod171/1 -> Mux/171
  "IW{1,1}(172,:)'"/1 -> dotprod172/1
  dotprod172/1 -> Mux/172
  "IW{1,1}(173,:)'"/1 -> dotprod173/1
  dotprod173/1 -> Mux/173
  "IW{1,1}(174,:)'"/1 -> dotprod174/1
  dotprod174/1 -> Mux/174
  "IW{1,1}(175,:)'"/1 -> dotprod175/1
  dotprod175/1 -> Mux/175
  "IW{1,1}(176,:)'"/1 -> dotprod176/1
  dotprod176/1 -> Mux/176
  "IW{1,1}(177,:)'"/1 -> dotprod177/1
  dotprod177/1 -> Mux/177
  "IW{1,1}(178,:)'"/1 -> dotprod178/1
  dotprod178/1 -> Mux/178
  "IW{1,1}(179,:)'"/1 -> dotprod179/1
  dotprod179/1 -> Mux/179
  "IW{1,1}(180,:)'"/1 -> dotprod180/1
  dotprod180/1 -> Mux/180
  "IW{1,1}(181,:)'"/1 -> dotprod181/1
  dotprod181/1 -> Mux/181
  "IW{1,1}(182,:)'"/1 -> dotprod182/1
  dotprod182/1 -> Mux/182
  "IW{1,1}(183,:)'"/1 -> dotprod183/1
  dotprod183/1 -> Mux/183
  "IW{1,1}(184,:)'"/1 -> dotprod184/1
  dotprod184/1 -> Mux/184
  "IW{1,1}(185,:)'"/1 -> dotprod185/1
  dotprod185/1 -> Mux/185
  "IW{1,1}(186,:)'"/1 -> dotprod186/1
  dotprod186/1 -> Mux/186
  "IW{1,1}(187,:)'"/1 -> dotprod187/1
  dotprod187/1 -> Mux/187
  "IW{1,1}(188,:)'"/1 -> dotprod188/1
  dotprod188/1 -> Mux/188
  "IW{1,1}(189,:)'"/1 -> dotprod189/1
  dotprod189/1 -> Mux/189
  "IW{1,1}(190,:)'"/1 -> dotprod190/1
  dotprod190/1 -> Mux/190
  "IW{1,1}(191,:)'"/1 -> dotprod191/1
  dotprod191/1 -> Mux/191
  "IW{1,1}(192,:)'"/1 -> dotprod192/1
  dotprod192/1 -> Mux/192
  "IW{1,1}(193,:)'"/1 -> dotprod193/1
  dotprod193/1 -> Mux/193
  "IW{1,1}(194,:)'"/1 -> dotprod194/1
  dotprod194/1 -> Mux/194
  "IW{1,1}(195,:)'"/1 -> dotprod195/1
  dotprod195/1 -> Mux/195
  "IW{1,1}(196,:)'"/1 -> dotprod196/1
  dotprod196/1 -> Mux/196
  "IW{1,1}(197,:)'"/1 -> dotprod197/1
  dotprod197/1 -> Mux/197
  "IW{1,1}(198,:)'"/1 -> dotprod198/1
  dotprod198/1 -> Mux/198
  "IW{1,1}(199,:)'"/1 -> dotprod199/1
  dotprod199/1 -> Mux/199
  "IW{1,1}(200,:)'"/1 -> dotprod200/1
  dotprod200/1 -> Mux/200
  Mux/1 -> "iz{1,1}"/1
